simulink library "outp"  (R2021b)
(part 5 of 7)

  VBCM_CountAlarm_enum_Inproc : FVT_lib/outp/OverrideAndLimit  SystemSampleTime=-1  VariantActivationTime=update diagram  Latency=0  AutoFrameSizeCalculation=off
      link override Signal_Limit/_maxval: Value=KOUTP_CountAlarm_enum_maxval
      link override Signal_Limit/_minval: Value=KOUTP_CountAlarm_enum_minval
      link override Signal_Override/_ovrdflg: Value=KOUTP_CountAlarm_enum_ovrdflg
      link override Signal_Override/_ovrdval: Value=KOUTP_CountAlarm_enum_ovrdval
  VBCM_CrashDetd_flg_Inproc : FVT_lib/outp/OverrideAndLimit  SystemSampleTime=-1  VariantActivationTime=update diagram  Latency=0  AutoFrameSizeCalculation=off
      link override Signal_Limit/_maxval: Value=KOUTP_CrashDetd_flg_maxval
      link override Signal_Limit/_minval: Value=KOUTP_CrashDetd_flg_minval
      link override Signal_Override/_ovrdflg: Value=KOUTP_CrashDetd_flg_ovrdflg
      link override Signal_Override/_ovrdval: Value=KOUTP_CrashDetd_flg_ovrdval
  VBCM_DimSwSta_flg_Inproc : FVT_lib/outp/OverrideAndLimit  SystemSampleTime=-1  VariantActivationTime=update diagram  Latency=0  AutoFrameSizeCalculation=off
      link override Signal_Limit/_maxval: Value=KOUTP_DimSwSta_flg_maxval
      link override Signal_Limit/_minval: Value=KOUTP_DimSwSta_flg_minval
      link override Signal_Override/_ovrdflg: Value=KOUTP_DimSwSta_flg_ovrdflg
      link override Signal_Override/_ovrdval: Value=KOUTP_DimSwSta_flg_ovrdval
  VBCM_DimmerEN_flg_Inproc : FVT_lib/outp/OverrideAndLimit  SystemSampleTime=-1  VariantActivationTime=update diagram  Latency=0  AutoFrameSizeCalculation=off
      link override Signal_Limit/_maxval: Value=KOUTP_DimmerEN_flg_maxval
      link override Signal_Limit/_minval: Value=KOUTP_DimmerEN_flg_minval
      link override Signal_Override/_ovrdflg: Value=KOUTP_DimmerEN_flg_ovrdflg
      link override Signal_Override/_ovrdval: Value=KOUTP_DimmerEN_flg_ovrdval
  VBCM_Dimmer_pct_Inproc : FVT_lib/outp/OverrideAndLimit  SystemSampleTime=-1  VariantActivationTime=update diagram  Latency=0  AutoFrameSizeCalculation=off
      link override Signal_Limit/_maxval: Value=KOUTP_Dimmer_pct_maxval
      link override Signal_Limit/_minval: Value=KOUTP_Dimmer_pct_minval
      link override Signal_Override/_ovrdflg: Value=KOUTP_Dimmer_pct_ovrdflg
      link override Signal_Override/_ovrdval: Value=KOUTP_Dimmer_pct_ovrdval
  VBCM_DoorLockIND_flg_Inproc : FVT_lib/outp/OverrideAndLimit  SystemSampleTime=-1  VariantActivationTime=update diagram  Latency=0  AutoFrameSizeCalculation=off
      link override Signal_Limit/_maxval: Value=KOUTP_DoorLockIND_flg_maxval
      link override Signal_Limit/_minval: Value=KOUTP_DoorLockIND_flg_minval
      link override Signal_Override/_ovrdflg: Value=KOUTP_DoorLockIND_flg_ovrdflg
      link override Signal_Override/_ovrdval: Value=KOUTP_DoorLockIND_flg_ovrdval
  VBCM_DrDoorSW_flg_Inproc : FVT_lib/outp/OverrideAndLimit  SystemSampleTime=-1  VariantActivationTime=update diagram  Latency=0  AutoFrameSizeCalculation=off
      link override Signal_Limit/_maxval: Value=KOUTP_DrDoorSW_flg_maxval
      link override Signal_Limit/_minval: Value=KOUTP_DrDoorSW_flg_minval
      link override Signal_Override/_ovrdflg: Value=KOUTP_DrDoorSW_flg_ovrdflg
      link override Signal_Override/_ovrdval: Value=KOUTP_DrDoorSW_flg_ovrdval
  VBCM_FWasSwSta_enum_Inproc : FVT_lib/outp/OverrideAndLimit  SystemSampleTime=-1  VariantActivationTime=update diagram  Latency=0  AutoFrameSizeCalculation=off
      link override Signal_Limit/_maxval: Value=KOUTP_FWasSwSta_enum_maxval
      link override Signal_Limit/_minval: Value=KOUTP_FWasSwSta_enum_minval
      link override Signal_Override/_ovrdflg: Value=KOUTP_FWasSwSta_enum_ovrdflg
      link override Signal_Override/_ovrdval: Value=KOUTP_FWasSwSta_enum_ovrdval
  VBCM_FWipSwSta_enum_Inproc : FVT_lib/outp/OverrideAndLimit  SystemSampleTime=-1  VariantActivationTime=update diagram  Latency=0  AutoFrameSizeCalculation=off
      link override Signal_Limit/_maxval: Value=KOUTP_FWipSwSta_enum_maxval
      link override Signal_Limit/_minval: Value=KOUTP_FWipSwSta_enum_minval
      link override Signal_Override/_ovrdflg: Value=KOUTP_FWipSwSta_enum_ovrdflg
      link override Signal_Override/_ovrdval: Value=KOUTP_FWipSwSta_enum_ovrdval
  VBCM_FollowMe_flg_Inproc : FVT_lib/outp/OverrideAndLimit  SystemSampleTime=-1  VariantActivationTime=update diagram  Latency=0  AutoFrameSizeCalculation=off
      link override Signal_Limit/_maxval: Value=KOUTP_FollowMe_flg_maxval
      link override Signal_Limit/_minval: Value=KOUTP_FollowMe_flg_minval
      link override Signal_Override/_ovrdflg: Value=KOUTP_FollowMe_flg_ovrdflg
      link override Signal_Override/_ovrdval: Value=KOUTP_FollowMe_flg_ovrdval
  VBCM_FrChargingDoorCtrl_enum_Inproc : FVT_lib/outp/OverrideAndLimit  SystemSampleTime=-1  VariantActivationTime=update diagram  Latency=0  AutoFrameSizeCalculation=off
      link override Signal_Limit/_maxval: Value=KOUTP_FrChargingDoorCtrl_enum_maxval
      link override Signal_Limit/_minval: Value=KOUTP_FrChargingDoorCtrl_enum_minval
      link override Signal_Override/_ovrdflg: Value=KOUTP_FrChargingDoorCtrl_enum_ovrdflg
      link override Signal_Override/_ovrdval: Value=KOUTP_FrChargingDoorCtrl_enum_ovrdval
  VBCM_FrWiperH_flg_Inproc : FVT_lib/outp/OverrideAndLimit  SystemSampleTime=-1  VariantActivationTime=update diagram  Latency=0  AutoFrameSizeCalculation=off
      link override Signal_Limit/_maxval: Value=KOUTP_FrWiperH_flg_maxval
      link override Signal_Limit/_minval: Value=KOUTP_FrWiperH_flg_minval
      link override Signal_Override/_ovrdflg: Value=KOUTP_FrWiperH_flg_ovrdflg
      link override Signal_Override/_ovrdval: Value=KOUTP_FrWiperH_flg_ovrdval
  VBCM_FrWiperL_flg_Inproc : FVT_lib/outp/OverrideAndLimit  SystemSampleTime=-1  VariantActivationTime=update diagram  Latency=0  AutoFrameSizeCalculation=off
      link override Signal_Limit/_maxval: Value=KOUTP_FrWiperL_flg_maxval
      link override Signal_Limit/_minval: Value=KOUTP_FrWiperL_flg_minval
      link override Signal_Override/_ovrdflg: Value=KOUTP_FrWiperL_flg_ovrdflg
      link override Signal_Override/_ovrdval: Value=KOUTP_FrWiperL_flg_ovrdval
  VBCM_FuelDoorPos_flg_Inproc : FVT_lib/outp/OverrideAndLimit  SystemSampleTime=-1  VariantActivationTime=update diagram  Latency=0  AutoFrameSizeCalculation=off
      link override Signal_Limit/_maxval: Value=KOUTP_FuelDoorPos_flg_maxval
      link override Signal_Limit/_minval: Value=KOUTP_FuelDoorPos_flg_minval
      link override Signal_Override/_ovrdflg: Value=KOUTP_FuelDoorPos_flg_ovrdflg
      link override Signal_Override/_ovrdval: Value=KOUTP_FuelDoorPos_flg_ovrdval
  VBCM_HBeam_flg_Inproc : FVT_lib/outp/OverrideAndLimit  SystemSampleTime=-1  VariantActivationTime=update diagram  Latency=0  AutoFrameSizeCalculation=off
      link override Signal_Limit/_maxval: Value=KOUTP_HBeam_flg_maxval
      link override Signal_Limit/_minval: Value=KOUTP_HBeam_flg_minval
      link override Signal_Override/_ovrdflg: Value=KOUTP_HBeam_flg_ovrdflg
      link override Signal_Override/_ovrdval: Value=KOUTP_HBeam_flg_ovrdval
  VBCM_HazardIND_flg_Inproc : FVT_lib/outp/OverrideAndLimit  SystemSampleTime=-1  VariantActivationTime=update diagram  Latency=0  AutoFrameSizeCalculation=off
      link override Signal_Limit/_maxval: Value=KOUTP_HazardIND_flg_maxval
      link override Signal_Limit/_minval: Value=KOUTP_HazardIND_flg_minval
      link override Signal_Override/_ovrdflg: Value=KOUTP_HazardIND_flg_ovrdflg
      link override Signal_Override/_ovrdval: Value=KOUTP_HazardIND_flg_ovrdval
  VBCM_HazardSW_flg_Inproc : FVT_lib/outp/OverrideAndLimit  SystemSampleTime=-1  VariantActivationTime=update diagram  Latency=0  AutoFrameSizeCalculation=off
      link override Signal_Limit/_maxval: Value=KOUTP_HazardSW_flg_maxval
      link override Signal_Limit/_minval: Value=KOUTP_HazardSW_flg_minval
      link override Signal_Override/_ovrdflg: Value=KOUTP_HazardSW_flg_ovrdflg
      link override Signal_Override/_ovrdval: Value=KOUTP_HazardSW_flg_ovrdval
  VBCM_HoodSW_flg_Inproc : FVT_lib/outp/OverrideAndLimit  SystemSampleTime=-1  VariantActivationTime=update diagram  Latency=0  AutoFrameSizeCalculation=off
      link override Signal_Limit/_maxval: Value=KOUTP_HoodSW_flg_maxval
      link override Signal_Limit/_minval: Value=KOUTP_HoodSW_flg_minval
      link override Signal_Override/_ovrdflg: Value=KOUTP_HoodSW_flg_ovrdflg
      link override Signal_Override/_ovrdval: Value=KOUTP_HoodSW_flg_ovrdval
  VBCM_HornCtrl_flg_Inproc : FVT_lib/outp/OverrideAndLimit  SystemSampleTime=-1  VariantActivationTime=update diagram  Latency=0  AutoFrameSizeCalculation=off
      link override Signal_Limit/_maxval: Value=KOUTP_HornCtrl_flg_maxval
      link override Signal_Limit/_minval: Value=KOUTP_HornCtrl_flg_minval
      link override Signal_Override/_ovrdflg: Value=KOUTP_HornCtrl_flg_ovrdflg
      link override Signal_Override/_ovrdval: Value=KOUTP_HornCtrl_flg_ovrdval
  VBCM_IVIPTGUSStaSW_flg_Inproc : FVT_lib/outp/OverrideAndLimit  SystemSampleTime=-1  VariantActivationTime=update diagram  Latency=0  AutoFrameSizeCalculation=off
      link override Signal_Limit/_maxval: Value=KOUTP_IVIPTGUSStaSW_flg_maxval
      link override Signal_Limit/_minval: Value=KOUTP_IVIPTGUSStaSW_flg_minval
      link override Signal_Override/_ovrdflg: Value=KOUTP_IVIPTGUSStaSW_flg_ovrdflg
      link override Signal_Override/_ovrdval: Value=KOUTP_IVIPTGUSStaSW_flg_ovrdval
  VBCM_IVIRST_flg_Inproc : FVT_lib/outp/OverrideAndLimit  SystemSampleTime=-1  VariantActivationTime=update diagram  Latency=0  AutoFrameSizeCalculation=off
      link override Signal_Limit/_maxval: Value=KOUTP_IVIRST_flg_maxval
      link override Signal_Limit/_minval: Value=KOUTP_IVIRST_flg_minval
      link override Signal_Override/_ovrdflg: Value=KOUTP_IVIRST_flg_ovrdflg
      link override Signal_Override/_ovrdval: Value=KOUTP_IVIRST_flg_ovrdval
  VBCM_LBSD_flg_Inproc : FVT_lib/outp/OverrideAndLimit  SystemSampleTime=-1  VariantActivationTime=update diagram  Latency=0  AutoFrameSizeCalculation=off
      link override Signal_Limit/_maxval: Value=KOUTP_LBSD_flg_maxval
      link override Signal_Limit/_minval: Value=KOUTP_LBSD_flg_minval
      link override Signal_Override/_ovrdflg: Value=KOUTP_LBSD_flg_ovrdflg
      link override Signal_Override/_ovrdval: Value=KOUTP_LBSD_flg_ovrdval
  VBCM_LBeam_flg_Inproc : FVT_lib/outp/OverrideAndLimit  SystemSampleTime=-1  VariantActivationTime=update diagram  Latency=0  AutoFrameSizeCalculation=off
      link override Signal_Limit/_maxval: Value=KOUTP_LBeam_flg_maxval
      link override Signal_Limit/_minval: Value=KOUTP_LBeam_flg_minval
      link override Signal_Override/_ovrdflg: Value=KOUTP_LBeam_flg_ovrdflg
      link override Signal_Override/_ovrdval: Value=KOUTP_LBeam_flg_ovrdval
  VBCM_LDRL_flg_Inproc : FVT_lib/outp/OverrideAndLimit  SystemSampleTime=-1  VariantActivationTime=update diagram  Latency=0  AutoFrameSizeCalculation=off
      link override Signal_Limit/_maxval: Value=KOUTP_LDRL_flg_maxval
      link override Signal_Limit/_minval: Value=KOUTP_LDRL_flg_minval
      link override Signal_Override/_ovrdflg: Value=KOUTP_LDRL_flg_ovrdflg
      link override Signal_Override/_ovrdval: Value=KOUTP_LDRL_flg_ovrdval
  VBCM_LDrvCtrlCmd_pct_Inproc : FVT_lib/outp/OverrideAndLimit  SystemSampleTime=-1  VariantActivationTime=update diagram  Latency=0  AutoFrameSizeCalculation=off
      link override Signal_Limit/_maxval: Value=KOUTP_LDrvCtrlCmd_pct_maxval
      link override Signal_Limit/_minval: Value=KOUTP_LDrvCtrlCmd_pct_minval
      link override Signal_Override/_ovrdflg: Value=KOUTP_LDrvCtrlCmd_pct_ovrdflg
      link override Signal_Override/_ovrdval: Value=KOUTP_LDrvCtrlCmd_pct_ovrdval
  VBCM_LPasCtrlCmd_pct_Inproc : FVT_lib/outp/OverrideAndLimit  SystemSampleTime=-1  VariantActivationTime=update diagram  Latency=0  AutoFrameSizeCalculation=off
      link override Signal_Limit/_maxval: Value=KOUTP_LPasCtrlCmd_pct_maxval
      link override Signal_Limit/_minval: Value=KOUTP_LPasCtrlCmd_pct_minval
      link override Signal_Override/_ovrdflg: Value=KOUTP_LPasCtrlCmd_pct_ovrdflg
      link override Signal_Override/_ovrdval: Value=KOUTP_LPasCtrlCmd_pct_ovrdval
  VBCM_LRLDCtrlCmd_pct_Inproc : FVT_lib/outp/OverrideAndLimit  SystemSampleTime=-1  VariantActivationTime=update diagram  Latency=0  AutoFrameSizeCalculation=off
      link override Signal_Limit/_maxval: Value=KOUTP_LRLDCtrlCmd_pct_maxval
      link override Signal_Limit/_minval: Value=KOUTP_LRLDCtrlCmd_pct_minval
      link override Signal_Override/_ovrdflg: Value=KOUTP_LRLDCtrlCmd_pct_ovrdflg
      link override Signal_Override/_ovrdval: Value=KOUTP_LRLDCtrlCmd_pct_ovrdval
  VBCM_LRRDCtrlCmd_pct_Inproc : FVT_lib/outp/OverrideAndLimit  SystemSampleTime=-1  VariantActivationTime=update diagram  Latency=0  AutoFrameSizeCalculation=off
      link override Signal_Limit/_maxval: Value=KOUTP_LRRDCtrlCmd_pct_maxval
      link override Signal_Limit/_minval: Value=KOUTP_LRRDCtrlCmd_pct_minval
      link override Signal_Override/_ovrdflg: Value=KOUTP_LRRDCtrlCmd_pct_ovrdflg
      link override Signal_Override/_ovrdval: Value=KOUTP_LRRDCtrlCmd_pct_ovrdval
  VBCM_LTurnLP_flg_Inproc : FVT_lib/outp/OverrideAndLimit  SystemSampleTime=-1  VariantActivationTime=update diagram  Latency=0  AutoFrameSizeCalculation=off
      link override Signal_Limit/_maxval: Value=KOUTP_LTurnLP_flg_maxval
      link override Signal_Limit/_minval: Value=KOUTP_LTurnLP_flg_minval
      link override Signal_Override/_ovrdflg: Value=KOUTP_LTurnLP_flg_ovrdflg
      link override Signal_Override/_ovrdval: Value=KOUTP_LTurnLP_flg_ovrdval
  VBCM_LampPwr_flg_Inproc : FVT_lib/outp/OverrideAndLimit  SystemSampleTime=-1  VariantActivationTime=update diagram  Latency=0  AutoFrameSizeCalculation=off
      link override Signal_Limit/_maxval: Value=KOUTP_LampPwr_flg_maxval
      link override Signal_Limit/_minval: Value=KOUTP_LampPwr_flg_minval
      link override Signal_Override/_ovrdflg: Value=KOUTP_LampPwr_flg_ovrdflg
      link override Signal_Override/_ovrdval: Value=KOUTP_LampPwr_flg_ovrdval
  VBCM_LockAlarm_enum_Inproc : FVT_lib/outp/OverrideAndLimit  SystemSampleTime=-1  VariantActivationTime=update diagram  Latency=0  AutoFrameSizeCalculation=off
      link override Signal_Limit/_maxval: Value=KOUTP_LockAlarm_enum_maxval
      link override Signal_Limit/_minval: Value=KOUTP_LockAlarm_enum_minval
      link override Signal_Override/_ovrdflg: Value=KOUTP_LockAlarm_enum_ovrdflg
      link override Signal_Override/_ovrdval: Value=KOUTP_LockAlarm_enum_ovrdval
  VBCM_LockSetting_flg_Inproc : FVT_lib/outp/OverrideAndLimit  SystemSampleTime=-1  VariantActivationTime=update diagram  Latency=0  AutoFrameSizeCalculation=off
      link override Signal_Limit/_maxval: Value=KOUTP_LockSetting_flg_maxval
      link override Signal_Limit/_minval: Value=KOUTP_LockSetting_flg_minval
      link override Signal_Override/_ovrdflg: Value=KOUTP_LockSetting_flg_ovrdflg
      link override Signal_Override/_ovrdval: Value=KOUTP_LockSetting_flg_ovrdval
  VBCM_MFRDNBrightReq_pct_Inproc : FVT_lib/outp/OverrideAndLimit  SystemSampleTime=-1  VariantActivationTime=update diagram  Latency=0  AutoFrameSizeCalculation=off
      link override Signal_Limit/_maxval: Value=KOUTP_MFRDNBrightReq_pct_maxval
      link override Signal_Limit/_minval: Value=KOUTP_MFRDNBrightReq_pct_minval
      link override Signal_Override/_ovrdflg: Value=KOUTP_MFRDNBrightReq_pct_ovrdflg
      link override Signal_Override/_ovrdval: Value=KOUTP_MFRDNBrightReq_pct_ovrdval
  VBCM_MFSWTri_flg_Inproc : FVT_lib/outp/OverrideAndLimit  SystemSampleTime=-1  VariantActivationTime=update diagram  Latency=0  AutoFrameSizeCalculation=off
      link override Signal_Limit/_maxval: Value=KOUTP_MFSWTri_flg_maxval
      link override Signal_Limit/_minval: Value=KOUTP_MFSWTri_flg_minval
      link override Signal_Override/_ovrdflg: Value=KOUTP_MFSWTri_flg_ovrdflg
      link override Signal_Override/_ovrdval: Value=KOUTP_MFSWTri_flg_ovrdval
  VBCM_MirrorCtrl_enum_Inproc : FVT_lib/outp/OverrideAndLimit  SystemSampleTime=-1  VariantActivationTime=update diagram  Latency=0  AutoFrameSizeCalculation=off
      link override Signal_Limit/_maxval: Value=KOUTP_MirrorCtrl_enum_maxval
      link override Signal_Limit/_minval: Value=KOUTP_MirrorCtrl_enum_minval
      link override Signal_Override/_ovrdflg: Value=KOUTP_MirrorCtrl_enum_ovrdflg
      link override Signal_Override/_ovrdval: Value=KOUTP_MirrorCtrl_enum_ovrdval
  VBCM_MirrorDefog_flg_Inproc : FVT_lib/outp/OverrideAndLimit  SystemSampleTime=-1  VariantActivationTime=update diagram  Latency=0  AutoFrameSizeCalculation=off
      link override Signal_Limit/_maxval: Value=KOUTP_MirrorDefog_flg_maxval
      link override Signal_Limit/_minval: Value=KOUTP_MirrorDefog_flg_minval
      link override Signal_Override/_ovrdflg: Value=KOUTP_MirrorDefog_flg_ovrdflg
      link override Signal_Override/_ovrdval: Value=KOUTP_MirrorDefog_flg_ovrdval
  VBCM_MirrorFlodPos_flg_Inproc : FVT_lib/outp/OverrideAndLimit  SystemSampleTime=-1  VariantActivationTime=update diagram  Latency=0  AutoFrameSizeCalculation=off
      link override Signal_Limit/_maxval: Value=KOUTP_MirrorFlodPos_flg_maxval
      link override Signal_Limit/_minval: Value=KOUTP_MirrorFlodPos_flg_minval
      link override Signal_Override/_ovrdflg: Value=KOUTP_MirrorFlodPos_flg_ovrdflg
      link override Signal_Override/_ovrdval: Value=KOUTP_MirrorFlodPos_flg_ovrdval
  VBCM_PTGInnerSW2_enum_Inproc : FVT_lib/outp/OverrideAndLimit  SystemSampleTime=-1  VariantActivationTime=update diagram  Latency=0  AutoFrameSizeCalculation=off
      link override Signal_Limit/_maxval: Value=KOUTP_PTGInnerSW2_enum_maxval
      link override Signal_Limit/_minval: Value=KOUTP_PTGInnerSW2_enum_minval
      link override Signal_Override/_ovrdflg: Value=KOUTP_PTGInnerSW2_enum_ovrdflg
      link override Signal_Override/_ovrdval: Value=KOUTP_PTGInnerSW2_enum_ovrdval
  VBCM_PassSWSta_flg_Inproc : FVT_lib/outp/OverrideAndLimit  SystemSampleTime=-1  VariantActivationTime=update diagram  Latency=0  AutoFrameSizeCalculation=off
      link override Signal_Limit/_maxval: Value=KOUTP_PassSWSta_flg_maxval
      link override Signal_Limit/_minval: Value=KOUTP_PassSWSta_flg_minval
      link override Signal_Override/_ovrdflg: Value=KOUTP_PassSWSta_flg_ovrdflg
      link override Signal_Override/_ovrdval: Value=KOUTP_PassSWSta_flg_ovrdval
  VBCM_PosLamp_flg_Inproc : FVT_lib/outp/OverrideAndLimit  SystemSampleTime=-1  VariantActivationTime=update diagram  Latency=0  AutoFrameSizeCalculation=off
      link override Signal_Limit/_maxval: Value=KOUTP_PosLamp_flg_maxval
      link override Signal_Limit/_minval: Value=KOUTP_PosLamp_flg_minval
      link override Signal_Override/_ovrdflg: Value=KOUTP_PosLamp_flg_ovrdflg
      link override Signal_Override/_ovrdval: Value=KOUTP_PosLamp_flg_ovrdval
  VBCM_PsDoorSW_flg_Inproc : FVT_lib/outp/OverrideAndLimit  SystemSampleTime=-1  VariantActivationTime=update diagram  Latency=0  AutoFrameSizeCalculation=off
      link override Signal_Limit/_maxval: Value=KOUTP_PsDoorSW_flg_maxval
      link override Signal_Limit/_minval: Value=KOUTP_PsDoorSW_flg_minval
      link override Signal_Override/_ovrdflg: Value=KOUTP_PsDoorSW_flg_ovrdflg
      link override Signal_Override/_ovrdval: Value=KOUTP_PsDoorSW_flg_ovrdval
  VBCM_RBSD_flg_Inproc : FVT_lib/outp/OverrideAndLimit  SystemSampleTime=-1  VariantActivationTime=update diagram  Latency=0  AutoFrameSizeCalculation=off
      link override Signal_Limit/_maxval: Value=KOUTP_RBSD_flg_maxval
      link override Signal_Limit/_minval: Value=KOUTP_RBSD_flg_minval
      link override Signal_Override/_ovrdflg: Value=KOUTP_RBSD_flg_ovrdflg
      link override Signal_Override/_ovrdval: Value=KOUTP_RBSD_flg_ovrdval
  VBCM_RDRL_flg_Inproc : FVT_lib/outp/OverrideAndLimit  SystemSampleTime=-1  VariantActivationTime=update diagram  Latency=0  AutoFrameSizeCalculation=off
      link override Signal_Limit/_maxval: Value=KOUTP_RDRL_flg_maxval
      link override Signal_Limit/_minval: Value=KOUTP_RDRL_flg_minval
      link override Signal_Override/_ovrdflg: Value=KOUTP_RDRL_flg_ovrdflg
      link override Signal_Override/_ovrdval: Value=KOUTP_RDRL_flg_ovrdval
  VBCM_RLDoorSW_flg_Inproc : FVT_lib/outp/OverrideAndLimit  SystemSampleTime=-1  VariantActivationTime=update diagram  Latency=0  AutoFrameSizeCalculation=off
      link override Signal_Limit/_maxval: Value=KOUTP_RLDoorSW_flg_maxval
      link override Signal_Limit/_minval: Value=KOUTP_RLDoorSW_flg_minval
      link override Signal_Override/_ovrdflg: Value=KOUTP_RLDoorSW_flg_ovrdflg
      link override Signal_Override/_ovrdval: Value=KOUTP_RLDoorSW_flg_ovrdval
  VBCM_RRDoorSW_flg_Inproc : FVT_lib/outp/OverrideAndLimit  SystemSampleTime=-1  VariantActivationTime=update diagram  Latency=0  AutoFrameSizeCalculation=off
      link override Signal_Limit/_maxval: Value=KOUTP_RRDoorSW_flg_maxval
      link override Signal_Limit/_minval: Value=KOUTP_RRDoorSW_flg_minval
      link override Signal_Override/_ovrdflg: Value=KOUTP_RRDoorSW_flg_ovrdflg
      link override Signal_Override/_ovrdval: Value=KOUTP_RRDoorSW_flg_ovrdval
  VBCM_RTurnLP_flg_Inproc : FVT_lib/outp/OverrideAndLimit  SystemSampleTime=-1  VariantActivationTime=update diagram  Latency=0  AutoFrameSizeCalculation=off
      link override Signal_Limit/_maxval: Value=KOUTP_RTurnLP_flg_maxval
      link override Signal_Limit/_minval: Value=KOUTP_RTurnLP_flg_minval
      link override Signal_Override/_ovrdflg: Value=KOUTP_RTurnLP_flg_ovrdflg
      link override Signal_Override/_ovrdval: Value=KOUTP_RTurnLP_flg_ovrdval
  VBCM_ReverseLamp_flg_Inproc : FVT_lib/outp/OverrideAndLimit  SystemSampleTime=-1  VariantActivationTime=update diagram  Latency=0  AutoFrameSizeCalculation=off
      link override Signal_Limit/_maxval: Value=KOUTP_ReverseLamp_flg_maxval
      link override Signal_Limit/_minval: Value=KOUTP_ReverseLamp_flg_minval
      link override Signal_Override/_ovrdflg: Value=KOUTP_ReverseLamp_flg_ovrdflg
      link override Signal_Override/_ovrdval: Value=KOUTP_ReverseLamp_flg_ovrdval
  VBCM_RoomLampH_flg_Inproc : FVT_lib/outp/OverrideAndLimit  SystemSampleTime=-1  VariantActivationTime=update diagram  Latency=0  AutoFrameSizeCalculation=off
      link override Signal_Limit/_maxval: Value=KOUTP_RoomLampH_flg_maxval
      link override Signal_Limit/_minval: Value=KOUTP_RoomLampH_flg_minval
      link override Signal_Override/_ovrdflg: Value=KOUTP_RoomLampH_flg_ovrdflg
      link override Signal_Override/_ovrdval: Value=KOUTP_RoomLampH_flg_ovrdval
  VBCM_RoomLampL_flg_Inproc : FVT_lib/outp/OverrideAndLimit  SystemSampleTime=-1  VariantActivationTime=update diagram  Latency=0  AutoFrameSizeCalculation=off
      link override Signal_Limit/_maxval: Value=KOUTP_RoomLampL_flg_maxval
      link override Signal_Limit/_minval: Value=KOUTP_RoomLampL_flg_minval
      link override Signal_Override/_ovrdflg: Value=KOUTP_RoomLampL_flg_ovrdflg
      link override Signal_Override/_ovrdval: Value=KOUTP_RoomLampL_flg_ovrdval
  VBCM_RoomLampMode_flg_Inproc : FVT_lib/outp/OverrideAndLimit  SystemSampleTime=-1  VariantActivationTime=update diagram  Latency=0  AutoFrameSizeCalculation=off
      link override Signal_Limit/_maxval: Value=KOUTP_RoomLampMode_flg_maxval
      link override Signal_Limit/_minval: Value=KOUTP_RoomLampMode_flg_minval
      link override Signal_Override/_ovrdflg: Value=KOUTP_RoomLampMode_flg_ovrdflg
      link override Signal_Override/_ovrdval: Value=KOUTP_RoomLampMode_flg_ovrdval
  VBCM_RrChargingDoorCtrl_enum_Inproc : FVT_lib/outp/OverrideAndLimit  SystemSampleTime=-1  VariantActivationTime=update diagram  Latency=0  AutoFrameSizeCalculation=off
      link override Signal_Limit/_maxval: Value=KOUTP_RrChargingDoorCtrl_enum_maxval
      link override Signal_Limit/_minval: Value=KOUTP_RrChargingDoorCtrl_enum_minval
      link override Signal_Override/_ovrdflg: Value=KOUTP_RrChargingDoorCtrl_enum_ovrdflg
      link override Signal_Override/_ovrdval: Value=KOUTP_RrChargingDoorCtrl_enum_ovrdval
  VBCM_RrDefog_flg_Inproc : FVT_lib/outp/OverrideAndLimit  SystemSampleTime=-1  VariantActivationTime=update diagram  Latency=0  AutoFrameSizeCalculation=off
      link override Signal_Limit/_maxval: Value=KOUTP_RrDefog_flg_maxval
      link override Signal_Limit/_minval: Value=KOUTP_RrDefog_flg_minval
      link override Signal_Override/_ovrdflg: Value=KOUTP_RrDefog_flg_ovrdflg
      link override Signal_Override/_ovrdval: Value=KOUTP_RrDefog_flg_ovrdval
  VBCM_RrFogLamp_flg_Inproc : FVT_lib/outp/OverrideAndLimit  SystemSampleTime=-1  VariantActivationTime=update diagram  Latency=0  AutoFrameSizeCalculation=off
      link override Signal_Limit/_maxval: Value=KOUTP_RrFogLamp_flg_maxval
      link override Signal_Limit/_minval: Value=KOUTP_RrFogLamp_flg_minval
      link override Signal_Override/_ovrdflg: Value=KOUTP_RrFogLamp_flg_ovrdflg
      link override Signal_Override/_ovrdval: Value=KOUTP_RrFogLamp_flg_ovrdval
  VBCM_RrWiper_flg_Inproc : FVT_lib/outp/OverrideAndLimit  SystemSampleTime=-1  VariantActivationTime=update diagram  Latency=0  AutoFrameSizeCalculation=off
      link override Signal_Limit/_maxval: Value=KOUTP_RrWiper_flg_maxval
      link override Signal_Limit/_minval: Value=KOUTP_RrWiper_flg_minval
      link override Signal_Override/_ovrdflg: Value=KOUTP_RrWiper_flg_ovrdflg
      link override Signal_Override/_ovrdval: Value=KOUTP_RrWiper_flg_ovrdval
  VBCM_SPTGDet_flg_Inproc : FVT_lib/outp/OverrideAndLimit  SystemSampleTime=-1  VariantActivationTime=update diagram  Latency=0  AutoFrameSizeCalculation=off
      link override Signal_Limit/_maxval: Value=KOUTP_SPTGDet_flg_maxval
      link override Signal_Limit/_minval: Value=KOUTP_SPTGDet_flg_minval
      link override Signal_Override/_ovrdflg: Value=KOUTP_SPTGDet_flg_ovrdflg
      link override Signal_Override/_ovrdval: Value=KOUTP_SPTGDet_flg_ovrdval
  VBCM_TailgateHDSW_flg_Inproc : FVT_lib/outp/OverrideAndLimit  SystemSampleTime=-1  VariantActivationTime=update diagram  Latency=0  AutoFrameSizeCalculation=off
      link override Signal_Limit/_maxval: Value=KOUTP_TailgateHDSW_flg_maxval
      link override Signal_Limit/_minval: Value=KOUTP_TailgateHDSW_flg_minval
      link override Signal_Override/_ovrdflg: Value=KOUTP_TailgateHDSW_flg_ovrdflg
      link override Signal_Override/_ovrdval: Value=KOUTP_TailgateHDSW_flg_ovrdval
  VBCM_TailgateRemote_enum_Inproc : FVT_lib/outp/OverrideAndLimit  SystemSampleTime=-1  VariantActivationTime=update diagram  Latency=0  AutoFrameSizeCalculation=off
      link override Signal_Limit/_maxval: Value=KOUTP_TailgateRemote_enum_maxval
      link override Signal_Limit/_minval: Value=KOUTP_TailgateRemote_enum_minval
      link override Signal_Override/_ovrdflg: Value=KOUTP_TailgateRemote_enum_ovrdflg
      link override Signal_Override/_ovrdval: Value=KOUTP_TailgateRemote_enum_ovrdval
  VBCM_TailgateSW_flg_Inproc : FVT_lib/outp/OverrideAndLimit  SystemSampleTime=-1  VariantActivationTime=update diagram  Latency=0  AutoFrameSizeCalculation=off
      link override Signal_Limit/_maxval: Value=KOUTP_TailgateSW_flg_maxval
      link override Signal_Limit/_minval: Value=KOUTP_TailgateSW_flg_minval
      link override Signal_Override/_ovrdflg: Value=KOUTP_TailgateSW_flg_ovrdflg
      link override Signal_Override/_ovrdval: Value=KOUTP_TailgateSW_flg_ovrdval
  VBCM_TrunkRel_flg_Inproc : FVT_lib/outp/OverrideAndLimit  SystemSampleTime=-1  VariantActivationTime=update diagram  Latency=0  AutoFrameSizeCalculation=off
      link override Signal_Limit/_maxval: Value=KOUTP_TrunkRel_flg_maxval
      link override Signal_Limit/_minval: Value=KOUTP_TrunkRel_flg_minval
      link override Signal_Override/_ovrdflg: Value=KOUTP_TrunkRel_flg_ovrdflg
      link override Signal_Override/_ovrdval: Value=KOUTP_TrunkRel_flg_ovrdval
  VBCM_TurnSwSta_enum_Inproc : FVT_lib/outp/OverrideAndLimit  SystemSampleTime=-1  VariantActivationTime=update diagram  Latency=0  AutoFrameSizeCalculation=off
      link override Signal_Limit/_maxval: Value=KOUTP_TurnSwSta_enum_maxval
      link override Signal_Limit/_minval: Value=KOUTP_TurnSwSta_enum_minval
      link override Signal_Override/_ovrdflg: Value=KOUTP_TurnSwSta_enum_ovrdflg
      link override Signal_Override/_ovrdval: Value=KOUTP_TurnSwSta_enum_ovrdval
  VBCM_UserNow_enum_Inproc : FVT_lib/outp/OverrideAndLimit  SystemSampleTime=-1  VariantActivationTime=update diagram  Latency=0  AutoFrameSizeCalculation=off
      link override Signal_Limit/_maxval: Value=KOUTP_UserNow_enum_maxval
      link override Signal_Limit/_minval: Value=KOUTP_UserNow_enum_minval
      link override Signal_Override/_ovrdflg: Value=KOUTP_UserNow_enum_ovrdflg
      link override Signal_Override/_ovrdval: Value=KOUTP_UserNow_enum_ovrdval
  VBCM_WasherCtrl_enum_Inproc : FVT_lib/outp/OverrideAndLimit  SystemSampleTime=-1  VariantActivationTime=update diagram  Latency=0  AutoFrameSizeCalculation=off
      link override Signal_Limit/_maxval: Value=KOUTP_WasherCtrl_enum_maxval
      link override Signal_Limit/_minval: Value=KOUTP_WasherCtrl_enum_minval
      link override Signal_Override/_ovrdflg: Value=KOUTP_WasherCtrl_enum_ovrdflg
      link override Signal_Override/_ovrdval: Value=KOUTP_WasherCtrl_enum_ovrdval
  VBCM_WiperFixMode_flg_Inproc : FVT_lib/outp/OverrideAndLimit  SystemSampleTime=-1  VariantActivationTime=update diagram  Latency=0  AutoFrameSizeCalculation=off
      link override Signal_Limit/_maxval: Value=KOUTP_WiperFixMode_flg_maxval
      link override Signal_Limit/_minval: Value=KOUTP_WiperFixMode_flg_minval
      link override Signal_Override/_ovrdflg: Value=KOUTP_WiperFixMode_flg_ovrdflg
      link override Signal_Override/_ovrdval: Value=KOUTP_WiperFixMode_flg_ovrdval
  VBCM_fUnlockSingle_flg_Inproc : FVT_lib/outp/OverrideAndLimit  SystemSampleTime=-1  VariantActivationTime=update diagram  Latency=0  AutoFrameSizeCalculation=off
      link override Signal_Limit/_maxval: Value=KOUTP_fUnlockSingle_flg_maxval
      link override Signal_Limit/_minval: Value=KOUTP_fUnlockSingle_flg_minval
      link override Signal_Override/_ovrdflg: Value=KOUTP_fUnlockSingle_flg_ovrdflg
      link override Signal_Override/_ovrdval: Value=KOUTP_fUnlockSingle_flg_ovrdval
  VDHP_ActAPSPosn_pct_Inproc : FVT_lib/outp/OverrideAndLimit  SystemSampleTime=-1  VariantActivationTime=update diagram  Latency=0  AutoFrameSizeCalculation=off
      link override Signal_Limit/_maxval: Value=KOUTP_ActAPSPosn_pct_maxval
      link override Signal_Limit/_minval: Value=KOUTP_ActAPSPosn_pct_minval
      link override Signal_Override/_ovrdflg: Value=KOUTP_ActAPSPosn_pct_ovrdflg
      link override Signal_Override/_ovrdval: Value=KOUTP_ActAPSPosn_pct_ovrdval
  VDHP_EAPS1MIN_pct_Inproc : FVT_lib/outp/OverrideAndLimit  SystemSampleTime=-1  VariantActivationTime=update diagram  Latency=0  AutoFrameSizeCalculation=off
      link override Signal_Limit/_maxval: Value=KOUTP_EAPS1MIN_pct_maxval
      link override Signal_Limit/_minval: Value=KOUTP_EAPS1MIN_pct_minval
      link override Signal_Override/_ovrdflg: Value=KOUTP_EAPS1MIN_pct_ovrdflg
      link override Signal_Override/_ovrdval: Value=KOUTP_EAPS1MIN_pct_ovrdval
  VDHP_EAPS2MIN_pct_Inproc : FVT_lib/outp/OverrideAndLimit  SystemSampleTime=-1  VariantActivationTime=update diagram  Latency=0  AutoFrameSizeCalculation=off
      link override Signal_Limit/_maxval: Value=KOUTP_EAPS2MIN_pct_maxval
      link override Signal_Limit/_minval: Value=KOUTP_EAPS2MIN_pct_minval
      link override Signal_Override/_ovrdflg: Value=KOUTP_EAPS2MIN_pct_ovrdflg
      link override Signal_Override/_ovrdval: Value=KOUTP_EAPS2MIN_pct_ovrdval
  VDKC_DKCAuthSta_enum_Inproc : FVT_lib/outp/OverrideAndLimit  SystemSampleTime=-1  VariantActivationTime=update diagram  Latency=0  AutoFrameSizeCalculation=off
      link override Signal_Limit/_maxval: Value=KOUTP_DKCAuthSta_enum_maxval
      link override Signal_Limit/_minval: Value=KOUTP_DKCAuthSta_enum_minval
      link override Signal_Override/_ovrdflg: Value=KOUTP_DKCAuthSta_enum_ovrdflg
      link override Signal_Override/_ovrdval: Value=KOUTP_DKCAuthSta_enum_ovrdval
  VDKC_DKCTimeSN_cnt_Inproc : FVT_lib/outp/OverrideAndLimit  SystemSampleTime=-1  VariantActivationTime=update diagram  Latency=0  AutoFrameSizeCalculation=off
      link override Signal_Limit/_maxval: Value=KOUTP_DKCTimeSN_cnt_maxval
      link override Signal_Limit/_minval: Value=KOUTP_DKCTimeSN_cnt_minval
      link override Signal_Override/_ovrdflg: Value=KOUTP_DKCTimeSN_cnt_ovrdflg
      link override Signal_Override/_ovrdval: Value=KOUTP_DKCTimeSN_cnt_ovrdval
  VDSC_DISCButtSta_flg_Inproc : FVT_lib/outp/OverrideAndLimit  SystemSampleTime=-1  VariantActivationTime=update diagram  Latency=0  AutoFrameSizeCalculation=off
      link override Signal_Limit/_maxval: Value=KOUTP_DISCButtSta_flg_maxval
      link override Signal_Limit/_minval: Value=KOUTP_DISCButtSta_flg_minval
      link override Signal_Override/_ovrdflg: Value=KOUTP_DISCButtSta_flg_ovrdflg
      link override Signal_Override/_ovrdval: Value=KOUTP_DISCButtSta_flg_ovrdval
  VDSC_DISCSta_enum_Inproc : FVT_lib/outp/OverrideAndLimit  SystemSampleTime=-1  VariantActivationTime=update diagram  Latency=0  AutoFrameSizeCalculation=off
      link override Signal_Limit/_maxval: Value=KOUTP_DISCSta_enum_maxval
      link override Signal_Limit/_minval: Value=KOUTP_DISCSta_enum_minval
      link override Signal_Override/_ovrdflg: Value=KOUTP_DISCSta_enum_ovrdflg
      link override Signal_Override/_ovrdval: Value=KOUTP_DISCSta_enum_ovrdval
  VDSC_DISCTargetSpd_kph_Inproc : FVT_lib/outp/OverrideAndLimit  SystemSampleTime=-1  VariantActivationTime=update diagram  Latency=0  AutoFrameSizeCalculation=off
      link override Signal_Limit/_maxval: Value=KOUTP_DISCTargetSpd_kph_maxval
      link override Signal_Limit/_minval: Value=KOUTP_DISCTargetSpd_kph_minval
      link override Signal_Override/_ovrdflg: Value=KOUTP_DISCTargetSpd_kph_ovrdflg
      link override Signal_Override/_ovrdval: Value=KOUTP_DISCTargetSpd_kph_ovrdval
  VDSC_DISCTurn_flg_Inproc : FVT_lib/outp/OverrideAndLimit  SystemSampleTime=-1  VariantActivationTime=update diagram  Latency=0  AutoFrameSizeCalculation=off
      link override Signal_Limit/_maxval: Value=KOUTP_DISCTurn_flg_maxval
      link override Signal_Limit/_minval: Value=KOUTP_DISCTurn_flg_minval
      link override Signal_Override/_ovrdflg: Value=KOUTP_DISCTurn_flg_ovrdflg
      link override Signal_Override/_ovrdval: Value=KOUTP_DISCTurn_flg_ovrdval
  VNMM_ActiveWU_flg_Inproc : FVT_lib/outp/OverrideAndLimit  SystemSampleTime=-1  VariantActivationTime=update diagram  Latency=0  AutoFrameSizeCalculation=off
      link override Signal_Limit/_maxval: Value=KOUTP_ActiveWU_flg_maxval
      link override Signal_Limit/_minval: Value=KOUTP_ActiveWU_flg_minval
      link override Signal_Override/_ovrdflg: Value=KOUTP_ActiveWU_flg_ovrdflg
      link override Signal_Override/_ovrdval: Value=KOUTP_ActiveWU_flg_ovrdval
  VNMM_AllCANTxReq_flg_Inproc : FVT_lib/outp/OverrideAndLimit  SystemSampleTime=-1  VariantActivationTime=update diagram  Latency=0  AutoFrameSizeCalculation=off
      link override Signal_Limit/_maxval: Value=KOUTP_AllCANTxReq_flg_maxval
      link override Signal_Limit/_minval: Value=KOUTP_AllCANTxReq_flg_minval
      link override Signal_Override/_ovrdflg: Value=KOUTP_AllCANTxReq_flg_ovrdflg
      link override Signal_Override/_ovrdval: Value=KOUTP_AllCANTxReq_flg_ovrdval
  VNMM_Awake_enum_Inproc : FVT_lib/outp/OverrideAndLimit  SystemSampleTime=-1  VariantActivationTime=update diagram  Latency=0  AutoFrameSizeCalculation=off
      link override Signal_Limit/_maxval: Value=KOUTP_Awake_enum_maxval
      link override Signal_Limit/_minval: Value=KOUTP_Awake_enum_minval
      link override Signal_Override/_ovrdflg: Value=KOUTP_Awake_enum_ovrdflg
      link override Signal_Override/_ovrdval: Value=KOUTP_Awake_enum_ovrdval
  VNMM_CSB_flg_Inproc : FVT_lib/outp/OverrideAndLimit  SystemSampleTime=-1  VariantActivationTime=update diagram  Latency=0  AutoFrameSizeCalculation=off
      link override Signal_Limit/_maxval: Value=KOUTP_CSB_flg_maxval
      link override Signal_Limit/_minval: Value=KOUTP_CSB_flg_minval
      link override Signal_Override/_ovrdflg: Value=KOUTP_CSB_flg_ovrdflg
      link override Signal_Override/_ovrdval: Value=KOUTP_CSB_flg_ovrdval
  VNMM_ErrorState_enum_Inproc : FVT_lib/outp/OverrideAndLimit  SystemSampleTime=-1  VariantActivationTime=update diagram  Latency=0  AutoFrameSizeCalculation=off
      link override Signal_Limit/_maxval: Value=KOUTP_ErrorState_enum_maxval
      link override Signal_Limit/_minval: Value=KOUTP_ErrorState_enum_minval
      link override Signal_Override/_ovrdflg: Value=KOUTP_ErrorState_enum_ovrdflg
      link override Signal_Override/_ovrdval: Value=KOUTP_ErrorState_enum_ovrdval
  VNMM_NMmTxReq_flg_Inproc : FVT_lib/outp/OverrideAndLimit  SystemSampleTime=-1  VariantActivationTime=update diagram  Latency=0  AutoFrameSizeCalculation=off
      link override Signal_Limit/_maxval: Value=KOUTP_NMmTxReq_flg_maxval
      link override Signal_Limit/_minval: Value=KOUTP_NMmTxReq_flg_minval
      link override Signal_Override/_ovrdflg: Value=KOUTP_NMmTxReq_flg_ovrdflg
      link override Signal_Override/_ovrdval: Value=KOUTP_NMmTxReq_flg_ovrdval
  VNMM_NetworkReq_flg_Inproc : FVT_lib/outp/OverrideAndLimit  SystemSampleTime=-1  VariantActivationTime=update diagram  Latency=0  AutoFrameSizeCalculation=off
      link override Signal_Limit/_maxval: Value=KOUTP_NetworkReq_flg_maxval
      link override Signal_Limit/_minval: Value=KOUTP_NetworkReq_flg_minval
      link override Signal_Override/_ovrdflg: Value=KOUTP_NetworkReq_flg_ovrdflg
      link override Signal_Override/_ovrdval: Value=KOUTP_NetworkReq_flg_ovrdval
  VNMM_NodeID_enum_Inproc : FVT_lib/outp/OverrideAndLimit  SystemSampleTime=-1  VariantActivationTime=update diagram  Latency=0  AutoFrameSizeCalculation=off
      link override Signal_Limit/_maxval: Value=KOUTP_NodeID_enum_maxval
      link override Signal_Limit/_minval: Value=KOUTP_NodeID_enum_minval
      link override Signal_Override/_ovrdflg: Value=KOUTP_NodeID_enum_ovrdflg
      link override Signal_Override/_ovrdval: Value=KOUTP_NodeID_enum_ovrdval
  VNMM_PNI_flg_Inproc : FVT_lib/outp/OverrideAndLimit  SystemSampleTime=-1  VariantActivationTime=update diagram  Latency=0  AutoFrameSizeCalculation=off
      link override Signal_Limit/_maxval: Value=KOUTP_PNI_flg_maxval
      link override Signal_Limit/_minval: Value=KOUTP_PNI_flg_minval
      link override Signal_Override/_ovrdflg: Value=KOUTP_PNI_flg_ovrdflg
      link override Signal_Override/_ovrdval: Value=KOUTP_PNI_flg_ovrdval
  VNMM_RptMsgReq_flg_Inproc : FVT_lib/outp/OverrideAndLimit  SystemSampleTime=-1  VariantActivationTime=update diagram  Latency=0  AutoFrameSizeCalculation=off
      link override Signal_Limit/_maxval: Value=KOUTP_RptMsgReq_flg_maxval
      link override Signal_Limit/_minval: Value=KOUTP_RptMsgReq_flg_minval
      link override Signal_Override/_ovrdflg: Value=KOUTP_RptMsgReq_flg_ovrdflg
      link override Signal_Override/_ovrdval: Value=KOUTP_RptMsgReq_flg_ovrdval
  VNMM_SysNMmSta_enum_Inproc : FVT_lib/outp/OverrideAndLimit  SystemSampleTime=-1  VariantActivationTime=update diagram  Latency=0  AutoFrameSizeCalculation=off
      link override Signal_Limit/_maxval: Value=KOUTP_SysNMmSta_enum_maxval
      link override Signal_Limit/_minval: Value=KOUTP_SysNMmSta_enum_minval
      link override Signal_Override/_ovrdflg: Value=KOUTP_SysNMmSta_enum_ovrdflg
      link override Signal_Override/_ovrdval: Value=KOUTP_SysNMmSta_enum_ovrdval
  VNMM_WakeUp_enum_Inproc : FVT_lib/outp/OverrideAndLimit  SystemSampleTime=-1  VariantActivationTime=update diagram  Latency=0  AutoFrameSizeCalculation=off
      link override Signal_Limit/_maxval: Value=KOUTP_WakeUp_enum_maxval
      link override Signal_Limit/_minval: Value=KOUTP_WakeUp_enum_minval
      link override Signal_Override/_ovrdflg: Value=KOUTP_WakeUp_enum_ovrdflg
      link override Signal_Override/_ovrdval: Value=KOUTP_WakeUp_enum_ovrdval
  VPMM_ActiveDischargeReq_flg_Inproc : FVT_lib/outp/OverrideAndLimit  SystemSampleTime=-1  VariantActivationTime=update diagram  Latency=0  AutoFrameSizeCalculation=off
      link override Signal_Limit/_maxval: Value=KOUTP_ActiveDischargeReq_flg_maxval
      link override Signal_Limit/_minval: Value=KOUTP_ActiveDischargeReq_flg_minval
      link override Signal_Override/_ovrdflg: Value=KOUTP_ActiveDischargeReq_flg_ovrdflg
      link override Signal_Override/_ovrdval: Value=KOUTP_ActiveDischargeReq_flg_ovrdval
  VPMM_CtrlDrPwrStbA2_flg_Inproc : FVT_lib/outp/OverrideAndLimit  SystemSampleTime=-1  VariantActivationTime=update diagram  Latency=0  AutoFrameSizeCalculation=off
      link override Signal_Limit/_maxval: Value=KOUTP_CtrlDrPwrStbA2_flg_maxval
      link override Signal_Limit/_minval: Value=KOUTP_CtrlDrPwrStbA2_flg_minval
      link override Signal_Override/_ovrdflg: Value=KOUTP_CtrlDrPwrStbA2_flg_ovrdflg
      link override Signal_Override/_ovrdval: Value=KOUTP_CtrlDrPwrStbA2_flg_ovrdval
  VPMM_CtrlFrBMSCCUCIR_flg_Inproc : FVT_lib/outp/OverrideAndLimit  SystemSampleTime=-1  VariantActivationTime=update diagram  Latency=0  AutoFrameSizeCalculation=off
      link override Signal_Limit/_maxval: Value=KOUTP_CtrlFrBMSCCUCIR_flg_maxval
      link override Signal_Limit/_minval: Value=KOUTP_CtrlFrBMSCCUCIR_flg_minval
      link override Signal_Override/_ovrdflg: Value=KOUTP_CtrlFrBMSCCUCIR_flg_ovrdflg
      link override Signal_Override/_ovrdval: Value=KOUTP_CtrlFrBMSCCUCIR_flg_ovrdval
  VPMM_CtrlFrEDUINVERTER_flg_Inproc : FVT_lib/outp/OverrideAndLimit  SystemSampleTime=-1  VariantActivationTime=update diagram  Latency=0  AutoFrameSizeCalculation=off
      link override Signal_Limit/_maxval: Value=KOUTP_CtrlFrEDUINVERTER_flg_maxval
      link override Signal_Limit/_minval: Value=KOUTP_CtrlFrEDUINVERTER_flg_minval
      link override Signal_Override/_ovrdflg: Value=KOUTP_CtrlFrEDUINVERTER_flg_ovrdflg
      link override Signal_Override/_ovrdval: Value=KOUTP_CtrlFrEDUINVERTER_flg_ovrdval
  VPMM_CtrlFrPwrStbA1P_flg_Inproc : FVT_lib/outp/OverrideAndLimit  SystemSampleTime=-1  VariantActivationTime=update diagram  Latency=0  AutoFrameSizeCalculation=off
      link override Signal_Limit/_maxval: Value=KOUTP_CtrlFrPwrStbA1P_flg_maxval
      link override Signal_Limit/_minval: Value=KOUTP_CtrlFrPwrStbA1P_flg_minval
      link override Signal_Override/_ovrdflg: Value=KOUTP_CtrlFrPwrStbA1P_flg_ovrdflg
      link override Signal_Override/_ovrdval: Value=KOUTP_CtrlFrPwrStbA1P_flg_ovrdval
  VPMM_CtrlFrRC1_flg_Inproc : FVT_lib/outp/OverrideAndLimit  SystemSampleTime=-1  VariantActivationTime=update diagram  Latency=0  AutoFrameSizeCalculation=off
      link override Signal_Limit/_maxval: Value=KOUTP_CtrlFrRC1_flg_maxval
      link override Signal_Limit/_minval: Value=KOUTP_CtrlFrRC1_flg_minval
      link override Signal_Override/_ovrdflg: Value=KOUTP_CtrlFrRC1_flg_ovrdflg
      link override Signal_Override/_ovrdval: Value=KOUTP_CtrlFrRC1_flg_ovrdval
  VPMM_DCDCEnaReq_flg_Inproc : FVT_lib/outp/OverrideAndLimit  SystemSampleTime=-1  VariantActivationTime=update diagram  Latency=0  AutoFrameSizeCalculation=off
      link override Signal_Limit/_maxval: Value=KOUTP_DCDCEnaReq_flg_maxval
      link override Signal_Limit/_minval: Value=KOUTP_DCDCEnaReq_flg_minval
      link override Signal_Override/_ovrdflg: Value=KOUTP_DCDCEnaReq_flg_ovrdflg
      link override Signal_Override/_ovrdval: Value=KOUTP_DCDCEnaReq_flg_ovrdval
  VPMM_DCDCVoltSetpoint_V_Inproc : FVT_lib/outp/OverrideAndLimit  SystemSampleTime=-1  VariantActivationTime=update diagram  Latency=0  AutoFrameSizeCalculation=off
      link override Signal_Limit/_maxval: Value=KOUTP_DCDCVoltSetpoint_V_maxval
      link override Signal_Limit/_minval: Value=KOUTP_DCDCVoltSetpoint_V_minval
      link override Signal_Override/_ovrdflg: Value=KOUTP_DCDCVoltSetpoint_V_ovrdflg
      link override Signal_Override/_ovrdval: Value=KOUTP_DCDCVoltSetpoint_V_ovrdval
  VPMM_DrSeatSta_enum_Inproc : FVT_lib/outp/OverrideAndLimit  SystemSampleTime=-1  VariantActivationTime=update diagram  Latency=0  AutoFrameSizeCalculation=off
      link override Signal_Limit/_maxval: Value=KOUTP_DrSeatSta_enum_maxval
      link override Signal_Limit/_minval: Value=KOUTP_DrSeatSta_enum_minval
      link override Signal_Override/_ovrdflg: Value=KOUTP_DrSeatSta_enum_ovrdflg
      link override Signal_Override/_ovrdval: Value=KOUTP_DrSeatSta_enum_ovrdval
  VPMM_DrivetrainSelect_enum_Inproc : FVT_lib/outp/OverrideAndLimit  SystemSampleTime=-1  VariantActivationTime=update diagram  Latency=0  AutoFrameSizeCalculation=off
      link override Signal_Limit/_maxval: Value=KOUTP_DrivetrainSelect_enum_maxval
      link override Signal_Limit/_minval: Value=KOUTP_DrivetrainSelect_enum_minval
      link override Signal_Override/_ovrdflg: Value=KOUTP_DrivetrainSelect_enum_ovrdflg
      link override Signal_Override/_ovrdval: Value=KOUTP_DrivetrainSelect_enum_ovrdval
  VPMM_EvccAplusPwrUpReq_flg_Inproc : FVT_lib/outp/OverrideAndLimit  SystemSampleTime=-1  VariantActivationTime=update diagram  Latency=0  AutoFrameSizeCalculation=off
      link override Signal_Limit/_maxval: Value=KOUTP_EvccAplusPwrUpReq_flg_maxval
      link override Signal_Limit/_minval: Value=KOUTP_EvccAplusPwrUpReq_flg_minval
      link override Signal_Override/_ovrdflg: Value=KOUTP_EvccAplusPwrUpReq_flg_ovrdflg
      link override Signal_Override/_ovrdval: Value=KOUTP_EvccAplusPwrUpReq_flg_ovrdval
  VPMM_FDADC12VDetAvg_mV_Inproc : FVT_lib/outp/OverrideAndLimit  SystemSampleTime=-1  VariantActivationTime=update diagram  Latency=0  AutoFrameSizeCalculation=off
      link override Signal_Limit/_maxval: Value=KOUTP_FDADC12VDetAvg_mV_maxval
      link override Signal_Limit/_minval: Value=KOUTP_FDADC12VDetAvg_mV_minval
      link override Signal_Override/_ovrdflg: Value=KOUTP_FDADC12VDetAvg_mV_ovrdflg
      link override Signal_Override/_ovrdval: Value=KOUTP_FDADC12VDetAvg_mV_ovrdval
  VPMM_FrMCUEnaReq_flg_Inproc : FVT_lib/outp/OverrideAndLimit  SystemSampleTime=-1  VariantActivationTime=update diagram  Latency=0  AutoFrameSizeCalculation=off
      link override Signal_Limit/_maxval: Value=KOUTP_FrMCUEnaReq_flg_maxval
      link override Signal_Limit/_minval: Value=KOUTP_FrMCUEnaReq_flg_minval
      link override Signal_Override/_ovrdflg: Value=KOUTP_FrMCUEnaReq_flg_ovrdflg
      link override Signal_Override/_ovrdval: Value=KOUTP_FrMCUEnaReq_flg_ovrdval
  VPMM_HVBatCnctReq_flg_Inproc : FVT_lib/outp/OverrideAndLimit  SystemSampleTime=-1  VariantActivationTime=update diagram  Latency=0  AutoFrameSizeCalculation=off
      link override Signal_Limit/_maxval: Value=KOUTP_HVBatCnctReq_flg_maxval
      link override Signal_Limit/_minval: Value=KOUTP_HVBatCnctReq_flg_minval
      link override Signal_Override/_ovrdflg: Value=KOUTP_HVBatCnctReq_flg_ovrdflg
      link override Signal_Override/_ovrdval: Value=KOUTP_HVBatCnctReq_flg_ovrdval
  VPMM_HVPwrSta_flg_Inproc : FVT_lib/outp/OverrideAndLimit  SystemSampleTime=-1  VariantActivationTime=update diagram  Latency=0  AutoFrameSizeCalculation=off
      link override Signal_Limit/_maxval: Value=KOUTP_HVPwrSta_flg_maxval
      link override Signal_Limit/_minval: Value=KOUTP_HVPwrSta_flg_minval
      link override Signal_Override/_ovrdflg: Value=KOUTP_HVPwrSta_flg_ovrdflg
      link override Signal_Override/_ovrdval: Value=KOUTP_HVPwrSta_flg_ovrdval
  VPMM_HVSysReadyToCharge_enum_Inproc : FVT_lib/outp/OverrideAndLimit  SystemSampleTime=-1  VariantActivationTime=update diagram  Latency=0  AutoFrameSizeCalculation=off
      link override Signal_Limit/_maxval: Value=KOUTP_HVSysReadyToCharge_enum_maxval
      link override Signal_Limit/_minval: Value=KOUTP_HVSysReadyToCharge_enum_minval
      link override Signal_Override/_ovrdflg: Value=KOUTP_HVSysReadyToCharge_enum_ovrdflg
      link override Signal_Override/_ovrdval: Value=KOUTP_HVSysReadyToCharge_enum_ovrdval
  VPMM_HWResetSta_enum_Inproc : FVT_lib/outp/OverrideAndLimit  SystemSampleTime=-1  VariantActivationTime=update diagram  Latency=0  AutoFrameSizeCalculation=off
      link override Signal_Limit/_maxval: Value=KOUTP_HWResetSta_enum_maxval
      link override Signal_Limit/_minval: Value=KOUTP_HWResetSta_enum_minval
      link override Signal_Override/_ovrdflg: Value=KOUTP_HWResetSta_enum_ovrdflg
      link override Signal_Override/_ovrdval: Value=KOUTP_HWResetSta_enum_ovrdval
  VPMM_IVIPwrStaONTOPopT_s_Inproc : FVT_lib/outp/OverrideAndLimit  SystemSampleTime=-1  VariantActivationTime=update diagram  Latency=0  AutoFrameSizeCalculation=off
      link override Signal_Limit/_maxval: Value=KOUTP_IVIPwrStaONTOPopT_s_maxval
      link override Signal_Limit/_minval: Value=KOUTP_IVIPwrStaONTOPopT_s_minval
      link override Signal_Override/_ovrdflg: Value=KOUTP_IVIPwrStaONTOPopT_s_ovrdflg
      link override Signal_Override/_ovrdval: Value=KOUTP_IVIPwrStaONTOPopT_s_ovrdval
  VPMM_LVBattChrgTimeCnt_s_Inproc : FVT_lib/outp/OverrideAndLimit  SystemSampleTime=-1  VariantActivationTime=update diagram  Latency=0  AutoFrameSizeCalculation=off
      link override Signal_Limit/_maxval: Value=KOUTP_LVBattChrgTimeCnt_s_maxval
      link override Signal_Limit/_minval: Value=KOUTP_LVBattChrgTimeCnt_s_minval
      link override Signal_Override/_ovrdflg: Value=KOUTP_LVBattChrgTimeCnt_s_ovrdflg
      link override Signal_Override/_ovrdval: Value=KOUTP_LVBattChrgTimeCnt_s_ovrdval
  VPMM_LVChrgHoldTtimer_s_Inproc : FVT_lib/outp/OverrideAndLimit  SystemSampleTime=-1  VariantActivationTime=update diagram  Latency=0  AutoFrameSizeCalculation=off
      link override Signal_Limit/_maxval: Value=KOUTP_LVChrgHoldTtimer_s_maxval
      link override Signal_Limit/_minval: Value=KOUTP_LVChrgHoldTtimer_s_minval
      link override Signal_Override/_ovrdflg: Value=KOUTP_LVChrgHoldTtimer_s_ovrdflg
      link override Signal_Override/_ovrdval: Value=KOUTP_LVChrgHoldTtimer_s_ovrdval
  VPMM_LVPwrSta_flg_Inproc : FVT_lib/outp/OverrideAndLimit  SystemSampleTime=-1  VariantActivationTime=update diagram  Latency=0  AutoFrameSizeCalculation=off
      link override Signal_Limit/_maxval: Value=KOUTP_LVPwrSta_flg_maxval
      link override Signal_Limit/_minval: Value=KOUTP_LVPwrSta_flg_minval
      link override Signal_Override/_ovrdflg: Value=KOUTP_LVPwrSta_flg_ovrdflg
      link override Signal_Override/_ovrdval: Value=KOUTP_LVPwrSta_flg_ovrdval
  VPMM_LVSilentChrgLv_enum_Inproc : FVT_lib/outp/OverrideAndLimit  SystemSampleTime=-1  VariantActivationTime=update diagram  Latency=0  AutoFrameSizeCalculation=off
      link override Signal_Limit/_maxval: Value=KOUTP_LVSilentChrgLv_enum_maxval
      link override Signal_Limit/_minval: Value=KOUTP_LVSilentChrgLv_enum_minval
      link override Signal_Override/_ovrdflg: Value=KOUTP_LVSilentChrgLv_enum_ovrdflg
      link override Signal_Override/_ovrdval: Value=KOUTP_LVSilentChrgLv_enum_ovrdval
  VPMM_LVSilentChrgReq_flg_Inproc : FVT_lib/outp/OverrideAndLimit  SystemSampleTime=-1  VariantActivationTime=update diagram  Latency=0  AutoFrameSizeCalculation=off
      link override Signal_Limit/_maxval: Value=KOUTP_LVSilentChrgReq_flg_maxval
      link override Signal_Limit/_minval: Value=KOUTP_LVSilentChrgReq_flg_minval
      link override Signal_Override/_ovrdflg: Value=KOUTP_LVSilentChrgReq_flg_ovrdflg
      link override Signal_Override/_ovrdval: Value=KOUTP_LVSilentChrgReq_flg_ovrdval
  VPMM_LVSilentChrgSta_enum_Inproc : FVT_lib/outp/OverrideAndLimit  SystemSampleTime=-1  VariantActivationTime=update diagram  Latency=0  AutoFrameSizeCalculation=off
      link override Signal_Limit/_maxval: Value=KOUTP_LVSilentChrgSta_enum_maxval
      link override Signal_Limit/_minval: Value=KOUTP_LVSilentChrgSta_enum_minval
      link override Signal_Override/_ovrdflg: Value=KOUTP_LVSilentChrgSta_enum_ovrdflg
      link override Signal_Override/_ovrdval: Value=KOUTP_LVSilentChrgSta_enum_ovrdval
  VPMM_LVSysErrPwrOutErr_flg_Inproc : FVT_lib/outp/OverrideAndLimit  SystemSampleTime=-1  VariantActivationTime=update diagram  Latency=0  AutoFrameSizeCalculation=off
      link override Signal_Limit/_maxval: Value=KOUTP_LVSysErrPwrOutErr_flg_maxval
      link override Signal_Limit/_minval: Value=KOUTP_LVSysErrPwrOutErr_flg_minval
      link override Signal_Override/_ovrdflg: Value=KOUTP_LVSysErrPwrOutErr_flg_ovrdflg
      link override Signal_Override/_ovrdval: Value=KOUTP_LVSysErrPwrOutErr_flg_ovrdval
  VPMM_LowSOCWarn_enum_Inproc : FVT_lib/outp/OverrideAndLimit  SystemSampleTime=-1  VariantActivationTime=update diagram  Latency=0  AutoFrameSizeCalculation=off
      link override Signal_Limit/_maxval: Value=KOUTP_LowSOCWarn_enum_maxval
      link override Signal_Limit/_minval: Value=KOUTP_LowSOCWarn_enum_minval
      link override Signal_Override/_ovrdflg: Value=KOUTP_LowSOCWarn_enum_ovrdflg
      link override Signal_Override/_ovrdval: Value=KOUTP_LowSOCWarn_enum_ovrdval
  VPMM_OTAPwrReqOFFChkSta_enum_Inproc : FVT_lib/outp/OverrideAndLimit  SystemSampleTime=-1  VariantActivationTime=update diagram  Latency=0  AutoFrameSizeCalculation=off
      link override Signal_Limit/_maxval: Value=KOUTP_OTAPwrReqOFFChkSta_enum_maxval
      link override Signal_Limit/_minval: Value=KOUTP_OTAPwrReqOFFChkSta_enum_minval
      link override Signal_Override/_ovrdflg: Value=KOUTP_OTAPwrReqOFFChkSta_enum_ovrdflg
      link override Signal_Override/_ovrdval: Value=KOUTP_OTAPwrReqOFFChkSta_enum_ovrdval
  VPMM_OTAPwrReqStdChkSta_enum_Inproc : FVT_lib/outp/OverrideAndLimit  SystemSampleTime=-1  VariantActivationTime=update diagram  Latency=0  AutoFrameSizeCalculation=off
      link override Signal_Limit/_maxval: Value=KOUTP_OTAPwrReqStdChkSta_enum_maxval
      link override Signal_Limit/_minval: Value=KOUTP_OTAPwrReqStdChkSta_enum_minval
      link override Signal_Override/_ovrdflg: Value=KOUTP_OTAPwrReqStdChkSta_enum_ovrdflg
      link override Signal_Override/_ovrdval: Value=KOUTP_OTAPwrReqStdChkSta_enum_ovrdval
  VPMM_PMMAllowECUSleep_flg_Inproc : FVT_lib/outp/OverrideAndLimit  SystemSampleTime=-1  VariantActivationTime=update diagram  Latency=0  AutoFrameSizeCalculation=off
      link override Signal_Limit/_maxval: Value=KOUTP_PMMAllowECUSleep_flg_maxval
      link override Signal_Limit/_minval: Value=KOUTP_PMMAllowECUSleep_flg_minval
      link override Signal_Override/_ovrdflg: Value=KOUTP_PMMAllowECUSleep_flg_ovrdflg
      link override Signal_Override/_ovrdval: Value=KOUTP_PMMAllowECUSleep_flg_ovrdval
  VPMM_PowerDownFault_enum_Inproc : FVT_lib/outp/OverrideAndLimit  SystemSampleTime=-1  VariantActivationTime=update diagram  Latency=0  AutoFrameSizeCalculation=off
      link override Signal_Limit/_maxval: Value=KOUTP_PowerDownFault_enum_maxval
      link override Signal_Limit/_minval: Value=KOUTP_PowerDownFault_enum_minval
      link override Signal_Override/_ovrdflg: Value=KOUTP_PowerDownFault_enum_ovrdflg
      link override Signal_Override/_ovrdval: Value=KOUTP_PowerDownFault_enum_ovrdval
  VPMM_PowerDownState_enum_Inproc : FVT_lib/outp/OverrideAndLimit  SystemSampleTime=-1  VariantActivationTime=update diagram  Latency=0  AutoFrameSizeCalculation=off
      link override Signal_Limit/_maxval: Value=KOUTP_PowerDownState_enum_maxval
      link override Signal_Limit/_minval: Value=KOUTP_PowerDownState_enum_minval
      link override Signal_Override/_ovrdflg: Value=KOUTP_PowerDownState_enum_ovrdflg
      link override Signal_Override/_ovrdval: Value=KOUTP_PowerDownState_enum_ovrdval
  VPMM_PowerSta_enum_Inproc : FVT_lib/outp/OverrideAndLimit  SystemSampleTime=-1  VariantActivationTime=update diagram  Latency=0  AutoFrameSizeCalculation=off
      link override Signal_Limit/_maxval: Value=KOUTP_PowerSta_enum_maxval
      link override Signal_Limit/_minval: Value=KOUTP_PowerSta_enum_minval
      link override Signal_Override/_ovrdflg: Value=KOUTP_PowerSta_enum_ovrdflg
      link override Signal_Override/_ovrdval: Value=KOUTP_PowerSta_enum_ovrdval
  VPMM_PowerUpFault_enum_Inproc : FVT_lib/outp/OverrideAndLimit  SystemSampleTime=-1  VariantActivationTime=update diagram  Latency=0  AutoFrameSizeCalculation=off
      link override Signal_Limit/_maxval: Value=KOUTP_PowerUpFault_enum_maxval
      link override Signal_Limit/_minval: Value=KOUTP_PowerUpFault_enum_minval
      link override Signal_Override/_ovrdflg: Value=KOUTP_PowerUpFault_enum_ovrdflg
      link override Signal_Override/_ovrdval: Value=KOUTP_PowerUpFault_enum_ovrdval
  VPMM_PowerUpState_enum_Inproc : FVT_lib/outp/OverrideAndLimit  SystemSampleTime=-1  VariantActivationTime=update diagram  Latency=0  AutoFrameSizeCalculation=off
      link override Signal_Limit/_maxval: Value=KOUTP_PowerUpState_enum_maxval
      link override Signal_Limit/_minval: Value=KOUTP_PowerUpState_enum_minval
      link override Signal_Override/_ovrdflg: Value=KOUTP_PowerUpState_enum_ovrdflg
      link override Signal_Override/_ovrdval: Value=KOUTP_PowerUpState_enum_ovrdval
  VPMM_PwrDownReq_enum_Inproc : FVT_lib/outp/OverrideAndLimit  SystemSampleTime=-1  VariantActivationTime=update diagram  Latency=0  AutoFrameSizeCalculation=off
      link override Signal_Limit/_maxval: Value=KOUTP_PwrDownReq_enum_maxval
      link override Signal_Limit/_minval: Value=KOUTP_PwrDownReq_enum_minval
      link override Signal_Override/_ovrdflg: Value=KOUTP_PwrDownReq_enum_ovrdflg
      link override Signal_Override/_ovrdval: Value=KOUTP_PwrDownReq_enum_ovrdval
  VPMM_PwrReq_OTA_enum_Inproc : FVT_lib/outp/OverrideAndLimit  SystemSampleTime=-1  VariantActivationTime=update diagram  Latency=0  AutoFrameSizeCalculation=off
      link override Signal_Limit/_maxval: Value=KOUTP_PwrReq_OTA_enum_maxval
      link override Signal_Limit/_minval: Value=KOUTP_PwrReq_OTA_enum_minval
      link override Signal_Override/_ovrdflg: Value=KOUTP_PwrReq_OTA_enum_ovrdflg
      link override Signal_Override/_ovrdval: Value=KOUTP_PwrReq_OTA_enum_ovrdval
  VPMM_PwrStaConstraint_enum_Inproc : FVT_lib/outp/OverrideAndLimit  SystemSampleTime=-1  VariantActivationTime=update diagram  Latency=0  AutoFrameSizeCalculation=off
      link override Signal_Limit/_maxval: Value=KOUTP_PwrStaConstraint_enum_maxval
      link override Signal_Limit/_minval: Value=KOUTP_PwrStaConstraint_enum_minval
      link override Signal_Override/_ovrdflg: Value=KOUTP_PwrStaConstraint_enum_ovrdflg
      link override Signal_Override/_ovrdval: Value=KOUTP_PwrStaConstraint_enum_ovrdval
  VPMM_PwrStaONTOPopReq_flg_Inproc : FVT_lib/outp/OverrideAndLimit  SystemSampleTime=-1  VariantActivationTime=update diagram  Latency=0  AutoFrameSizeCalculation=off
      link override Signal_Limit/_maxval: Value=KOUTP_PwrStaONTOPopReq_flg_maxval
      link override Signal_Limit/_minval: Value=KOUTP_PwrStaONTOPopReq_flg_minval
      link override Signal_Override/_ovrdflg: Value=KOUTP_PwrStaONTOPopReq_flg_ovrdflg
      link override Signal_Override/_ovrdval: Value=KOUTP_PwrStaONTOPopReq_flg_ovrdval
  VPMM_PwrStaSelect_enum_Inproc : FVT_lib/outp/OverrideAndLimit  SystemSampleTime=-1  VariantActivationTime=update diagram  Latency=0  AutoFrameSizeCalculation=off
      link override Signal_Limit/_maxval: Value=KOUTP_PwrStaSelect_enum_maxval
      link override Signal_Limit/_minval: Value=KOUTP_PwrStaSelect_enum_minval
      link override Signal_Override/_ovrdflg: Value=KOUTP_PwrStaSelect_enum_ovrdflg
      link override Signal_Override/_ovrdval: Value=KOUTP_PwrStaSelect_enum_ovrdval
  VPMM_PwrStaTOSta_enum_Inproc : FVT_lib/outp/OverrideAndLimit  SystemSampleTime=-1  VariantActivationTime=update diagram  Latency=0  AutoFrameSizeCalculation=off
      link override Signal_Limit/_maxval: Value=KOUTP_PwrStaTOSta_enum_maxval
      link override Signal_Limit/_minval: Value=KOUTP_PwrStaTOSta_enum_minval
      link override Signal_Override/_ovrdflg: Value=KOUTP_PwrStaTOSta_enum_ovrdflg
      link override Signal_Override/_ovrdval: Value=KOUTP_PwrStaTOSta_enum_ovrdval
  VPMM_PwrUpReq_enum_Inproc : FVT_lib/outp/OverrideAndLimit  SystemSampleTime=-1  VariantActivationTime=update diagram  Latency=0  AutoFrameSizeCalculation=off
      link override Signal_Limit/_maxval: Value=KOUTP_PwrUpReq_enum_maxval
      link override Signal_Limit/_minval: Value=KOUTP_PwrUpReq_enum_minval
      link override Signal_Override/_ovrdflg: Value=KOUTP_PwrUpReq_enum_ovrdflg
      link override Signal_Override/_ovrdval: Value=KOUTP_PwrUpReq_enum_ovrdval
  VPMM_ReVehThdChkSta_enum_Inproc : FVT_lib/outp/OverrideAndLimit  SystemSampleTime=-1  VariantActivationTime=update diagram  Latency=0  AutoFrameSizeCalculation=off
      link override Signal_Limit/_maxval: Value=KOUTP_ReVehThdChkSta_enum_maxval
      link override Signal_Limit/_minval: Value=KOUTP_ReVehThdChkSta_enum_minval
      link override Signal_Override/_ovrdflg: Value=KOUTP_ReVehThdChkSta_enum_ovrdflg
      link override Signal_Override/_ovrdval: Value=KOUTP_ReVehThdChkSta_enum_ovrdval
  VPMM_RrMCUEnaReq_flg_Inproc : FVT_lib/outp/OverrideAndLimit  SystemSampleTime=-1  VariantActivationTime=update diagram  Latency=0  AutoFrameSizeCalculation=off
      link override Signal_Limit/_maxval: Value=KOUTP_RrMCUEnaReq_flg_maxval
      link override Signal_Limit/_minval: Value=KOUTP_RrMCUEnaReq_flg_minval
      link override Signal_Override/_ovrdflg: Value=KOUTP_RrMCUEnaReq_flg_ovrdflg
      link override Signal_Override/_ovrdval: Value=KOUTP_RrMCUEnaReq_flg_ovrdval
  VPMM_Sched_ChgTOSta_enum_Inproc : FVT_lib/outp/OverrideAndLimit  SystemSampleTime=-1  VariantActivationTime=update diagram  Latency=0  AutoFrameSizeCalculation=off
      link override Signal_Limit/_maxval: Value=KOUTP_Sched_ChgTOSta_enum_maxval
      link override Signal_Limit/_minval: Value=KOUTP_Sched_ChgTOSta_enum_minval
      link override Signal_Override/_ovrdflg: Value=KOUTP_Sched_ChgTOSta_enum_ovrdflg
      link override Signal_Override/_ovrdval: Value=KOUTP_Sched_ChgTOSta_enum_ovrdval
  VPMM_SilentChkAllowSleep_flg_Inproc : FVT_lib/outp/OverrideAndLimit  SystemSampleTime=-1  VariantActivationTime=update diagram  Latency=0  AutoFrameSizeCalculation=off
      link override Signal_Limit/_maxval: Value=KOUTP_SilentChkAllowSleep_flg_maxval
      link override Signal_Limit/_minval: Value=KOUTP_SilentChkAllowSleep_flg_minval
      link override Signal_Override/_ovrdflg: Value=KOUTP_SilentChkAllowSleep_flg_ovrdflg
      link override Signal_Override/_ovrdval: Value=KOUTP_SilentChkAllowSleep_flg_ovrdval
  VPMM_SysPowerMode_enum_Inproc : FVT_lib/outp/OverrideAndLimit  SystemSampleTime=-1  VariantActivationTime=update diagram  Latency=0  AutoFrameSizeCalculation=off
      link override Signal_Limit/_maxval: Value=KOUTP_SysPowerMode_enum_maxval
      link override Signal_Limit/_minval: Value=KOUTP_SysPowerMode_enum_minval
      link override Signal_Override/_ovrdflg: Value=KOUTP_SysPowerMode_enum_ovrdflg
      link override Signal_Override/_ovrdval: Value=KOUTP_SysPowerMode_enum_ovrdval
  VPMM_TCountSta_enum_Inproc : FVT_lib/outp/OverrideAndLimit  SystemSampleTime=-1  VariantActivationTime=update diagram  Latency=0  AutoFrameSizeCalculation=off
      link override Signal_Limit/_maxval: Value=KOUTP_TCountSta_enum_maxval
      link override Signal_Limit/_minval: Value=KOUTP_TCountSta_enum_minval
      link override Signal_Override/_ovrdflg: Value=KOUTP_TCountSta_enum_ovrdflg
      link override Signal_Override/_ovrdval: Value=KOUTP_TCountSta_enum_ovrdval
  VPMM_TimerAllowSleep_flg_Inproc : FVT_lib/outp/OverrideAndLimit  SystemSampleTime=-1  VariantActivationTime=update diagram  Latency=0  AutoFrameSizeCalculation=off
      link override Signal_Limit/_maxval: Value=KOUTP_TimerAllowSleep_flg_maxval
      link override Signal_Limit/_minval: Value=KOUTP_TimerAllowSleep_flg_minval
      link override Signal_Override/_ovrdflg: Value=KOUTP_TimerAllowSleep_flg_ovrdflg
      link override Signal_Override/_ovrdval: Value=KOUTP_TimerAllowSleep_flg_ovrdval
  VSYS_AcoreRebootCmdACK_flg_Inproc : FVT_lib/outp/OverrideAndLimit  SystemSampleTime=-1  VariantActivationTime=update diagram  Latency=0  AutoFrameSizeCalculation=off
      link override Signal_Limit/_maxval: Value=KOUTP_AcoreRebootCmdACK_flg_maxval
      link override Signal_Limit/_minval: Value=KOUTP_AcoreRebootCmdACK_flg_minval
      link override Signal_Override/_ovrdflg: Value=KOUTP_AcoreRebootCmdACK_flg_ovrdflg
      link override Signal_Override/_ovrdval: Value=KOUTP_AcoreRebootCmdACK_flg_ovrdval
  VSYS_CarModel1_cnt_Inproc : FVT_lib/outp/OverrideAndLimit  SystemSampleTime=-1  VariantActivationTime=update diagram  Latency=0  AutoFrameSizeCalculation=off
      link override Signal_Limit/_maxval: Value=KOUTP_CarModel1_cnt_maxval
      link override Signal_Limit/_minval: Value=KOUTP_CarModel1_cnt_minval
      link override Signal_Override/_ovrdflg: Value=KOUTP_CarModel1_cnt_ovrdflg
      link override Signal_Override/_ovrdval: Value=KOUTP_CarModel1_cnt_ovrdval
  VSYS_CarModel2_cnt_Inproc : FVT_lib/outp/OverrideAndLimit  SystemSampleTime=-1  VariantActivationTime=update diagram  Latency=0  AutoFrameSizeCalculation=off
      link override Signal_Limit/_maxval: Value=KOUTP_CarModel2_cnt_maxval
      link override Signal_Limit/_minval: Value=KOUTP_CarModel2_cnt_minval
      link override Signal_Override/_ovrdflg: Value=KOUTP_CarModel2_cnt_ovrdflg
      link override Signal_Override/_ovrdval: Value=KOUTP_CarModel2_cnt_ovrdval
  VSYS_CarModel3_cnt_Inproc : FVT_lib/outp/OverrideAndLimit  SystemSampleTime=-1  VariantActivationTime=update diagram  Latency=0  AutoFrameSizeCalculation=off
      link override Signal_Limit/_maxval: Value=KOUTP_CarModel3_cnt_maxval
      link override Signal_Limit/_minval: Value=KOUTP_CarModel3_cnt_minval
      link override Signal_Override/_ovrdflg: Value=KOUTP_CarModel3_cnt_ovrdflg
      link override Signal_Override/_ovrdval: Value=KOUTP_CarModel3_cnt_ovrdval
  VSYS_Change1_cnt_Inproc : FVT_lib/outp/OverrideAndLimit  SystemSampleTime=-1  VariantActivationTime=update diagram  Latency=0  AutoFrameSizeCalculation=off
      link override Signal_Limit/_maxval: Value=KOUTP_Change1_cnt_maxval
      link override Signal_Limit/_minval: Value=KOUTP_Change1_cnt_minval
      link override Signal_Override/_ovrdflg: Value=KOUTP_Change1_cnt_ovrdflg
      link override Signal_Override/_ovrdval: Value=KOUTP_Change1_cnt_ovrdval
  VSYS_Change2_cnt_Inproc : FVT_lib/outp/OverrideAndLimit  SystemSampleTime=-1  VariantActivationTime=update diagram  Latency=0  AutoFrameSizeCalculation=off
      link override Signal_Limit/_maxval: Value=KOUTP_Change2_cnt_maxval
      link override Signal_Limit/_minval: Value=KOUTP_Change2_cnt_minval
      link override Signal_Override/_ovrdflg: Value=KOUTP_Change2_cnt_ovrdflg
      link override Signal_Override/_ovrdval: Value=KOUTP_Change2_cnt_ovrdval
  VSYS_Country1_cnt_Inproc : FVT_lib/outp/OverrideAndLimit  SystemSampleTime=-1  VariantActivationTime=update diagram  Latency=0  AutoFrameSizeCalculation=off
      link override Signal_Limit/_maxval: Value=KOUTP_Country1_cnt_maxval
      link override Signal_Limit/_minval: Value=KOUTP_Country1_cnt_minval
      link override Signal_Override/_ovrdflg: Value=KOUTP_Country1_cnt_ovrdflg
      link override Signal_Override/_ovrdval: Value=KOUTP_Country1_cnt_ovrdval
  VSYS_Country2_cnt_Inproc : FVT_lib/outp/OverrideAndLimit  SystemSampleTime=-1  VariantActivationTime=update diagram  Latency=0  AutoFrameSizeCalculation=off
      link override Signal_Limit/_maxval: Value=KOUTP_Country2_cnt_maxval
      link override Signal_Limit/_minval: Value=KOUTP_Country2_cnt_minval
      link override Signal_Override/_ovrdflg: Value=KOUTP_Country2_cnt_ovrdflg
      link override Signal_Override/_ovrdval: Value=KOUTP_Country2_cnt_ovrdval
  VSYS_CurrentNmState_enum_Inproc : FVT_lib/outp/OverrideAndLimit  SystemSampleTime=-1  VariantActivationTime=update diagram  Latency=0  AutoFrameSizeCalculation=off
      link override Signal_Limit/_maxval: Value=KOUTP_CurrentNmState_enum_maxval
      link override Signal_Limit/_minval: Value=KOUTP_CurrentNmState_enum_minval
      link override Signal_Override/_ovrdflg: Value=KOUTP_CurrentNmState_enum_ovrdflg
      link override Signal_Override/_ovrdval: Value=KOUTP_CurrentNmState_enum_ovrdval
  VSYS_Dash1_cnt_Inproc : FVT_lib/outp/OverrideAndLimit  SystemSampleTime=-1  VariantActivationTime=update diagram  Latency=0  AutoFrameSizeCalculation=off
      link override Signal_Limit/_maxval: Value=KOUTP_Dash1_cnt_maxval
      link override Signal_Limit/_minval: Value=KOUTP_Dash1_cnt_minval
      link override Signal_Override/_ovrdflg: Value=KOUTP_Dash1_cnt_ovrdflg
      link override Signal_Override/_ovrdval: Value=KOUTP_Dash1_cnt_ovrdval
  VSYS_Dash2_cnt_Inproc : FVT_lib/outp/OverrideAndLimit  SystemSampleTime=-1  VariantActivationTime=update diagram  Latency=0  AutoFrameSizeCalculation=off
      link override Signal_Limit/_maxval: Value=KOUTP_Dash2_cnt_maxval
      link override Signal_Limit/_minval: Value=KOUTP_Dash2_cnt_minval
      link override Signal_Override/_ovrdflg: Value=KOUTP_Dash2_cnt_ovrdflg
      link override Signal_Override/_ovrdval: Value=KOUTP_Dash2_cnt_ovrdval
  VSYS_ECU1_cnt_Inproc : FVT_lib/outp/OverrideAndLimit  SystemSampleTime=-1  VariantActivationTime=update diagram  Latency=0  AutoFrameSizeCalculation=off
      link override Signal_Limit/_maxval: Value=KOUTP_ECU1_cnt_maxval
      link override Signal_Limit/_minval: Value=KOUTP_ECU1_cnt_minval
      link override Signal_Override/_ovrdflg: Value=KOUTP_ECU1_cnt_ovrdflg
      link override Signal_Override/_ovrdval: Value=KOUTP_ECU1_cnt_ovrdval
  VSYS_ECU2_cnt_Inproc : FVT_lib/outp/OverrideAndLimit  SystemSampleTime=-1  VariantActivationTime=update diagram  Latency=0  AutoFrameSizeCalculation=off
      link override Signal_Limit/_maxval: Value=KOUTP_ECU2_cnt_maxval
      link override Signal_Limit/_minval: Value=KOUTP_ECU2_cnt_minval
      link override Signal_Override/_ovrdflg: Value=KOUTP_ECU2_cnt_ovrdflg
      link override Signal_Override/_ovrdval: Value=KOUTP_ECU2_cnt_ovrdval
  VSYS_FdcSlpReqRisingEdge_flg_Inproc : FVT_lib/outp/OverrideAndLimit  SystemSampleTime=-1  VariantActivationTime=update diagram  Latency=0  AutoFrameSizeCalculation=off
      link override Signal_Limit/_maxval: Value=KOUTP_FdcSlpReqRisingEdge_flg_maxval
      link override Signal_Limit/_minval: Value=KOUTP_FdcSlpReqRisingEdge_flg_minval
      link override Signal_Override/_ovrdflg: Value=KOUTP_FdcSlpReqRisingEdge_flg_ovrdflg
      link override Signal_Override/_ovrdval: Value=KOUTP_FdcSlpReqRisingEdge_flg_ovrdval
  VSYS_FdcSlpTime_sec_Inproc : FVT_lib/outp/OverrideAndLimit  SystemSampleTime=-1  VariantActivationTime=update diagram  Latency=0  AutoFrameSizeCalculation=off
      link override Signal_Limit/_maxval: Value=KOUTP_FdcSlpTime_sec_maxval
      link override Signal_Limit/_minval: Value=KOUTP_FdcSlpTime_sec_minval
      link override Signal_Override/_ovrdflg: Value=KOUTP_FdcSlpTime_sec_ovrdflg
      link override Signal_Override/_ovrdval: Value=KOUTP_FdcSlpTime_sec_ovrdval
  VSYS_HWVer1_cnt_Inproc : FVT_lib/outp/OverrideAndLimit  SystemSampleTime=-1  VariantActivationTime=update diagram  Latency=0  AutoFrameSizeCalculation=off
      link override Signal_Limit/_maxval: Value=KOUTP_HWVer1_cnt_maxval
      link override Signal_Limit/_minval: Value=KOUTP_HWVer1_cnt_minval
      link override Signal_Override/_ovrdflg: Value=KOUTP_HWVer1_cnt_ovrdflg
      link override Signal_Override/_ovrdval: Value=KOUTP_HWVer1_cnt_ovrdval
  VSYS_HWVer2_cnt_Inproc : FVT_lib/outp/OverrideAndLimit  SystemSampleTime=-1  VariantActivationTime=update diagram  Latency=0  AutoFrameSizeCalculation=off
      link override Signal_Limit/_maxval: Value=KOUTP_HWVer2_cnt_maxval
      link override Signal_Limit/_minval: Value=KOUTP_HWVer2_cnt_minval
      link override Signal_Override/_ovrdflg: Value=KOUTP_HWVer2_cnt_ovrdflg
      link override Signal_Override/_ovrdval: Value=KOUTP_HWVer2_cnt_ovrdval
  VSYS_HWVer3_cnt_Inproc : FVT_lib/outp/OverrideAndLimit  SystemSampleTime=-1  VariantActivationTime=update diagram  Latency=0  AutoFrameSizeCalculation=off
      link override Signal_Limit/_maxval: Value=KOUTP_HWVer3_cnt_maxval
      link override Signal_Limit/_minval: Value=KOUTP_HWVer3_cnt_minval
      link override Signal_Override/_ovrdflg: Value=KOUTP_HWVer3_cnt_ovrdflg
      link override Signal_Override/_ovrdval: Value=KOUTP_HWVer3_cnt_ovrdval
  VSYS_Major1_cnt_Inproc : FVT_lib/outp/OverrideAndLimit  SystemSampleTime=-1  VariantActivationTime=update diagram  Latency=0  AutoFrameSizeCalculation=off
      link override Signal_Limit/_maxval: Value=KOUTP_Major1_cnt_maxval
      link override Signal_Limit/_minval: Value=KOUTP_Major1_cnt_minval
      link override Signal_Override/_ovrdflg: Value=KOUTP_Major1_cnt_ovrdflg
      link override Signal_Override/_ovrdval: Value=KOUTP_Major1_cnt_ovrdval
  VSYS_Major2_cnt_Inproc : FVT_lib/outp/OverrideAndLimit  SystemSampleTime=-1  VariantActivationTime=update diagram  Latency=0  AutoFrameSizeCalculation=off
      link override Signal_Limit/_maxval: Value=KOUTP_Major2_cnt_maxval
      link override Signal_Limit/_minval: Value=KOUTP_Major2_cnt_minval
      link override Signal_Override/_ovrdflg: Value=KOUTP_Major2_cnt_ovrdflg
      link override Signal_Override/_ovrdval: Value=KOUTP_Major2_cnt_ovrdval
  VSYS_Minor1_cnt_Inproc : FVT_lib/outp/OverrideAndLimit  SystemSampleTime=-1  VariantActivationTime=update diagram  Latency=0  AutoFrameSizeCalculation=off
      link override Signal_Limit/_maxval: Value=KOUTP_Minor1_cnt_maxval
      link override Signal_Limit/_minval: Value=KOUTP_Minor1_cnt_minval
      link override Signal_Override/_ovrdflg: Value=KOUTP_Minor1_cnt_ovrdflg
      link override Signal_Override/_ovrdval: Value=KOUTP_Minor1_cnt_ovrdval
  VSYS_Minor2_cnt_Inproc : FVT_lib/outp/OverrideAndLimit  SystemSampleTime=-1  VariantActivationTime=update diagram  Latency=0  AutoFrameSizeCalculation=off
      link override Signal_Limit/_maxval: Value=KOUTP_Minor2_cnt_maxval
      link override Signal_Limit/_minval: Value=KOUTP_Minor2_cnt_minval
      link override Signal_Override/_ovrdflg: Value=KOUTP_Minor2_cnt_ovrdflg
      link override Signal_Override/_ovrdval: Value=KOUTP_Minor2_cnt_ovrdval
  VSYS_NvWriteReqRisingEdge_flg_Inproc : FVT_lib/outp/OverrideAndLimit  SystemSampleTime=-1  VariantActivationTime=update diagram  Latency=0  AutoFrameSizeCalculation=off
      link override Signal_Limit/_maxval: Value=KOUTP_NvWriteReqRisingEdge_flg_maxval
      link override Signal_Limit/_minval: Value=KOUTP_NvWriteReqRisingEdge_flg_minval
      link override Signal_Override/_ovrdflg: Value=KOUTP_NvWriteReqRisingEdge_flg_ovrdflg
      link override Signal_Override/_ovrdval: Value=KOUTP_NvWriteReqRisingEdge_flg_ovrdval
  VSYS_Patch1_cnt_Inproc : FVT_lib/outp/OverrideAndLimit  SystemSampleTime=-1  VariantActivationTime=update diagram  Latency=0  AutoFrameSizeCalculation=off
      link override Signal_Limit/_maxval: Value=KOUTP_Patch1_cnt_maxval
      link override Signal_Limit/_minval: Value=KOUTP_Patch1_cnt_minval
      link override Signal_Override/_ovrdflg: Value=KOUTP_Patch1_cnt_ovrdflg
      link override Signal_Override/_ovrdval: Value=KOUTP_Patch1_cnt_ovrdval
  VSYS_Patch2_cnt_Inproc : FVT_lib/outp/OverrideAndLimit  SystemSampleTime=-1  VariantActivationTime=update diagram  Latency=0  AutoFrameSizeCalculation=off
      link override Signal_Limit/_maxval: Value=KOUTP_Patch2_cnt_maxval
      link override Signal_Limit/_minval: Value=KOUTP_Patch2_cnt_minval
      link override Signal_Override/_ovrdflg: Value=KOUTP_Patch2_cnt_ovrdflg
      link override Signal_Override/_ovrdval: Value=KOUTP_Patch2_cnt_ovrdval
  VSYS_PmicBootReason_enum_Inproc : FVT_lib/outp/OverrideAndLimit  SystemSampleTime=-1  VariantActivationTime=update diagram  Latency=0  AutoFrameSizeCalculation=off
      link override Signal_Limit/_maxval: Value=KOUTP_PmicBootReason_enum_maxval
      link override Signal_Limit/_minval: Value=KOUTP_PmicBootReason_enum_minval
      link override Signal_Override/_ovrdflg: Value=KOUTP_PmicBootReason_enum_ovrdflg
      link override Signal_Override/_ovrdval: Value=KOUTP_PmicBootReason_enum_ovrdval
  VSYS_SHA1_cnt_Inproc : FVT_lib/outp/OverrideAndLimit  SystemSampleTime=-1  VariantActivationTime=update diagram  Latency=0  AutoFrameSizeCalculation=off
      link override Signal_Limit/_maxval: Value=KOUTP_SHA1_cnt_maxval
      link override Signal_Limit/_minval: Value=KOUTP_SHA1_cnt_minval
      link override Signal_Override/_ovrdflg: Value=KOUTP_SHA1_cnt_ovrdflg
      link override Signal_Override/_ovrdval: Value=KOUTP_SHA1_cnt_ovrdval
  VSYS_SHA2_cnt_Inproc : FVT_lib/outp/OverrideAndLimit  SystemSampleTime=-1  VariantActivationTime=update diagram  Latency=0  AutoFrameSizeCalculation=off
      link override Signal_Limit/_maxval: Value=KOUTP_SHA2_cnt_maxval
      link override Signal_Limit/_minval: Value=KOUTP_SHA2_cnt_minval
      link override Signal_Override/_ovrdflg: Value=KOUTP_SHA2_cnt_ovrdflg
      link override Signal_Override/_ovrdval: Value=KOUTP_SHA2_cnt_ovrdval
  VSYS_SHA3_cnt_Inproc : FVT_lib/outp/OverrideAndLimit  SystemSampleTime=-1  VariantActivationTime=update diagram  Latency=0  AutoFrameSizeCalculation=off
      link override Signal_Limit/_maxval: Value=KOUTP_SHA3_cnt_maxval
      link override Signal_Limit/_minval: Value=KOUTP_SHA3_cnt_minval
      link override Signal_Override/_ovrdflg: Value=KOUTP_SHA3_cnt_ovrdflg
      link override Signal_Override/_ovrdval: Value=KOUTP_SHA3_cnt_ovrdval
  VSYS_SHA4_cnt_Inproc : FVT_lib/outp/OverrideAndLimit  SystemSampleTime=-1  VariantActivationTime=update diagram  Latency=0  AutoFrameSizeCalculation=off
      link override Signal_Limit/_maxval: Value=KOUTP_SHA4_cnt_maxval
      link override Signal_Limit/_minval: Value=KOUTP_SHA4_cnt_minval
      link override Signal_Override/_ovrdflg: Value=KOUTP_SHA4_cnt_ovrdflg
      link override Signal_Override/_ovrdval: Value=KOUTP_SHA4_cnt_ovrdval
  VSYS_SHA5_cnt_Inproc : FVT_lib/outp/OverrideAndLimit  SystemSampleTime=-1  VariantActivationTime=update diagram  Latency=0  AutoFrameSizeCalculation=off
      link override Signal_Limit/_maxval: Value=KOUTP_SHA5_cnt_maxval
      link override Signal_Limit/_minval: Value=KOUTP_SHA5_cnt_minval
      link override Signal_Override/_ovrdflg: Value=KOUTP_SHA5_cnt_ovrdflg
      link override Signal_Override/_ovrdval: Value=KOUTP_SHA5_cnt_ovrdval
  VSYS_SHA6_cnt_Inproc : FVT_lib/outp/OverrideAndLimit  SystemSampleTime=-1  VariantActivationTime=update diagram  Latency=0  AutoFrameSizeCalculation=off
      link override Signal_Limit/_maxval: Value=KOUTP_SHA6_cnt_maxval
      link override Signal_Limit/_minval: Value=KOUTP_SHA6_cnt_minval
      link override Signal_Override/_ovrdflg: Value=KOUTP_SHA6_cnt_ovrdflg
      link override Signal_Override/_ovrdval: Value=KOUTP_SHA6_cnt_ovrdval
  VSYS_SHA7_cnt_Inproc : FVT_lib/outp/OverrideAndLimit  SystemSampleTime=-1  VariantActivationTime=update diagram  Latency=0  AutoFrameSizeCalculation=off
      link override Signal_Limit/_maxval: Value=KOUTP_SHA7_cnt_maxval
      link override Signal_Limit/_minval: Value=KOUTP_SHA7_cnt_minval
      link override Signal_Override/_ovrdflg: Value=KOUTP_SHA7_cnt_ovrdflg
      link override Signal_Override/_ovrdval: Value=KOUTP_SHA7_cnt_ovrdval
  VSYS_SHA8_cnt_Inproc : FVT_lib/outp/OverrideAndLimit  SystemSampleTime=-1  VariantActivationTime=update diagram  Latency=0  AutoFrameSizeCalculation=off
      link override Signal_Limit/_maxval: Value=KOUTP_SHA8_cnt_maxval
      link override Signal_Limit/_minval: Value=KOUTP_SHA8_cnt_minval
      link override Signal_Override/_ovrdflg: Value=KOUTP_SHA8_cnt_ovrdflg
      link override Signal_Override/_ovrdval: Value=KOUTP_SHA8_cnt_ovrdval
  VSYS_Variation_cnt_Inproc : FVT_lib/outp/OverrideAndLimit  SystemSampleTime=-1  VariantActivationTime=update diagram  Latency=0  AutoFrameSizeCalculation=off
      link override Signal_Limit/_maxval: Value=KOUTP_Variation_cnt_maxval
      link override Signal_Limit/_minval: Value=KOUTP_Variation_cnt_minval
      link override Signal_Override/_ovrdflg: Value=KOUTP_Variation_cnt_ovrdflg
      link override Signal_Override/_ovrdval: Value=KOUTP_Variation_cnt_ovrdval
  VSYS_WisrBootReason_raw32_Inproc : FVT_lib/outp/OverrideAndLimit  SystemSampleTime=-1  VariantActivationTime=update diagram  Latency=0  AutoFrameSizeCalculation=off
      link override Signal_Limit/_maxval: Value=KOUTP_WisrBootReason_raw32_maxval
      link override Signal_Limit/_minval: Value=KOUTP_WisrBootReason_raw32_minval
      link override Signal_Override/_ovrdflg: Value=KOUTP_WisrBootReason_raw32_ovrdflg
      link override Signal_Override/_ovrdval: Value=KOUTP_WisrBootReason_raw32_ovrdval
  VTHC_ACForceOFF_flg_Inproc : FVT_lib/outp/OverrideAndLimit  SystemSampleTime=-1  VariantActivationTime=update diagram  Latency=0  AutoFrameSizeCalculation=off
      link override Signal_Limit/_maxval: Value=KOUTP_ACForceOFF_flg_maxval
      link override Signal_Limit/_minval: Value=KOUTP_ACForceOFF_flg_minval
      link override Signal_Override/_ovrdflg: Value=KOUTP_ACForceOFF_flg_ovrdflg
      link override Signal_Override/_ovrdval: Value=KOUTP_ACForceOFF_flg_ovrdval
  VTHC_ACModeMem_enum_Inproc : FVT_lib/outp/OverrideAndLimit  SystemSampleTime=-1  VariantActivationTime=update diagram  Latency=0  AutoFrameSizeCalculation=off
      link override Signal_Limit/_maxval: Value=KOUTP_ACModeMem_enum_maxval
      link override Signal_Limit/_minval: Value=KOUTP_ACModeMem_enum_minval
      link override Signal_Override/_ovrdflg: Value=KOUTP_ACModeMem_enum_ovrdflg
      link override Signal_Override/_ovrdval: Value=KOUTP_ACModeMem_enum_ovrdval
  VTHC_ACSubMode_enum_Inproc : FVT_lib/outp/OverrideAndLimit  SystemSampleTime=-1  VariantActivationTime=update diagram  Latency=0  AutoFrameSizeCalculation=off
      link override Signal_Limit/_maxval: Value=KOUTP_ACSubMode_enum_maxval
      link override Signal_Limit/_minval: Value=KOUTP_ACSubMode_enum_minval
      link override Signal_Override/_ovrdflg: Value=KOUTP_ACSubMode_enum_ovrdflg
      link override Signal_Override/_ovrdval: Value=KOUTP_ACSubMode_enum_ovrdval
  VTHC_AirIntenZone1M_enum_Inproc : FVT_lib/outp/OverrideAndLimit  SystemSampleTime=-1  VariantActivationTime=update diagram  Latency=0  AutoFrameSizeCalculation=off
      link override Signal_Limit/_maxval: Value=KOUTP_AirIntenZone1M_enum_maxval
      link override Signal_Limit/_minval: Value=KOUTP_AirIntenZone1M_enum_minval
      link override Signal_Override/_ovrdflg: Value=KOUTP_AirIntenZone1M_enum_ovrdflg
      link override Signal_Override/_ovrdval: Value=KOUTP_AirIntenZone1M_enum_ovrdval
  VTHC_BatteryMode_enum_Inproc : FVT_lib/outp/OverrideAndLimit  SystemSampleTime=-1  VariantActivationTime=update diagram  Latency=0  AutoFrameSizeCalculation=off
      link override Signal_Limit/_maxval: Value=KOUTP_BatteryMode_enum_maxval
      link override Signal_Limit/_minval: Value=KOUTP_BatteryMode_enum_minval
      link override Signal_Override/_ovrdflg: Value=KOUTP_BatteryMode_enum_ovrdflg
      link override Signal_Override/_ovrdval: Value=KOUTP_BatteryMode_enum_ovrdval
  VTHC_CCUACLampSts_flg_Inproc : FVT_lib/outp/OverrideAndLimit  SystemSampleTime=-1  VariantActivationTime=update diagram  Latency=0  AutoFrameSizeCalculation=off
      link override Signal_Limit/_maxval: Value=KOUTP_CCUACLampSts_flg_maxval
      link override Signal_Limit/_minval: Value=KOUTP_CCUACLampSts_flg_minval
      link override Signal_Override/_ovrdflg: Value=KOUTP_CCUACLampSts_flg_ovrdflg
      link override Signal_Override/_ovrdval: Value=KOUTP_CCUACLampSts_flg_ovrdval
  VTHC_CCUACMaxLampSts_flg_Inproc : FVT_lib/outp/OverrideAndLimit  SystemSampleTime=-1  VariantActivationTime=update diagram  Latency=0  AutoFrameSizeCalculation=off
      link override Signal_Limit/_maxval: Value=KOUTP_CCUACMaxLampSts_flg_maxval
      link override Signal_Limit/_minval: Value=KOUTP_CCUACMaxLampSts_flg_minval
      link override Signal_Override/_ovrdflg: Value=KOUTP_CCUACMaxLampSts_flg_ovrdflg
      link override Signal_Override/_ovrdval: Value=KOUTP_CCUACMaxLampSts_flg_ovrdval
  VTHC_CCUAutoLampSts_flg_Inproc : FVT_lib/outp/OverrideAndLimit  SystemSampleTime=-1  VariantActivationTime=update diagram  Latency=0  AutoFrameSizeCalculation=off
      link override Signal_Limit/_maxval: Value=KOUTP_CCUAutoLampSts_flg_maxval
      link override Signal_Limit/_minval: Value=KOUTP_CCUAutoLampSts_flg_minval
      link override Signal_Override/_ovrdflg: Value=KOUTP_CCUAutoLampSts_flg_ovrdflg
      link override Signal_Override/_ovrdval: Value=KOUTP_CCUAutoLampSts_flg_ovrdval
  VTHC_CCUSyncLampSts_flg_Inproc : FVT_lib/outp/OverrideAndLimit  SystemSampleTime=-1  VariantActivationTime=update diagram  Latency=0  AutoFrameSizeCalculation=off
      link override Signal_Limit/_maxval: Value=KOUTP_CCUSyncLampSts_flg_maxval
      link override Signal_Limit/_minval: Value=KOUTP_CCUSyncLampSts_flg_minval
      link override Signal_Override/_ovrdflg: Value=KOUTP_CCUSyncLampSts_flg_ovrdflg
      link override Signal_Override/_ovrdval: Value=KOUTP_CCUSyncLampSts_flg_ovrdval
  VTHC_CCUSyncSts_flg_Inproc : FVT_lib/outp/OverrideAndLimit  SystemSampleTime=-1  VariantActivationTime=update diagram  Latency=0  AutoFrameSizeCalculation=off
      link override Signal_Limit/_maxval: Value=KOUTP_CCUSyncSts_flg_maxval
      link override Signal_Limit/_minval: Value=KOUTP_CCUSyncSts_flg_minval
      link override Signal_Override/_ovrdflg: Value=KOUTP_CCUSyncSts_flg_ovrdflg
      link override Signal_Override/_ovrdval: Value=KOUTP_CCUSyncSts_flg_ovrdval
  VTHC_CabinMode_enum_Inproc : FVT_lib/outp/OverrideAndLimit  SystemSampleTime=-1  VariantActivationTime=update diagram  Latency=0  AutoFrameSizeCalculation=off
      link override Signal_Limit/_maxval: Value=KOUTP_CabinMode_enum_maxval
      link override Signal_Limit/_minval: Value=KOUTP_CabinMode_enum_minval
      link override Signal_Override/_ovrdflg: Value=KOUTP_CabinMode_enum_ovrdflg
      link override Signal_Override/_ovrdval: Value=KOUTP_CabinMode_enum_ovrdval
  VTHC_CoolgFanActDuty_pct_Inproc : FVT_lib/outp/OverrideAndLimit  SystemSampleTime=-1  VariantActivationTime=update diagram  Latency=0  AutoFrameSizeCalculation=off
      link override Signal_Limit/_maxval: Value=KOUTP_CoolgFanActDuty_pct_maxval
      link override Signal_Limit/_minval: Value=KOUTP_CoolgFanActDuty_pct_minval
      link override Signal_Override/_ovrdflg: Value=KOUTP_CoolgFanActDuty_pct_ovrdflg
      link override Signal_Override/_ovrdval: Value=KOUTP_CoolgFanActDuty_pct_ovrdval
  VTHC_EDriveMode_enum_Inproc : FVT_lib/outp/OverrideAndLimit  SystemSampleTime=-1  VariantActivationTime=update diagram  Latency=0  AutoFrameSizeCalculation=off
      link override Signal_Limit/_maxval: Value=KOUTP_EDriveMode_enum_maxval
      link override Signal_Limit/_minval: Value=KOUTP_EDriveMode_enum_minval
      link override Signal_Override/_ovrdflg: Value=KOUTP_EDriveMode_enum_ovrdflg
      link override Signal_Override/_ovrdval: Value=KOUTP_EDriveMode_enum_ovrdval
  VTHC_FDAGSCmd_enum_Inproc : FVT_lib/outp/OverrideAndLimit  SystemSampleTime=-1  VariantActivationTime=update diagram  Latency=0  AutoFrameSizeCalculation=off
      link override Signal_Limit/_maxval: Value=KOUTP_FDAGSCmd_enum_maxval
      link override Signal_Limit/_minval: Value=KOUTP_FDAGSCmd_enum_minval
      link override Signal_Override/_ovrdflg: Value=KOUTP_FDAGSCmd_enum_ovrdflg
      link override Signal_Override/_ovrdval: Value=KOUTP_FDAGSCmd_enum_ovrdval
  VTHC_FDBlowerCmd_pct_Inproc : FVT_lib/outp/OverrideAndLimit  SystemSampleTime=-1  VariantActivationTime=update diagram  Latency=0  AutoFrameSizeCalculation=off
      link override Signal_Limit/_maxval: Value=KOUTP_FDBlowerCmd_pct_maxval
      link override Signal_Limit/_minval: Value=KOUTP_FDBlowerCmd_pct_minval
      link override Signal_Override/_ovrdflg: Value=KOUTP_FDBlowerCmd_pct_ovrdflg
      link override Signal_Override/_ovrdval: Value=KOUTP_FDBlowerCmd_pct_ovrdval
  VTHC_FDCTHCMAPTCWarningSta_flg_Inproc : FVT_lib/outp/OverrideAndLimit  SystemSampleTime=-1  VariantActivationTime=update diagram  Latency=0  AutoFrameSizeCalculation=off
      link override Signal_Limit/_maxval: Value=KOUTP_FDCTHCMAPTCWarningSta_flg_maxval
      link override Signal_Limit/_minval: Value=KOUTP_FDCTHCMAPTCWarningSta_flg_minval
      link override Signal_Override/_ovrdflg: Value=KOUTP_FDCTHCMAPTCWarningSta_flg_ovrdflg
      link override Signal_Override/_ovrdval: Value=KOUTP_FDCTHCMAPTCWarningSta_flg_ovrdval
  VTHC_FDCompCmd_rpm_Inproc : FVT_lib/outp/OverrideAndLimit  SystemSampleTime=-1  VariantActivationTime=update diagram  Latency=0  AutoFrameSizeCalculation=off
      link override Signal_Limit/_maxval: Value=KOUTP_FDCompCmd_rpm_maxval
      link override Signal_Limit/_minval: Value=KOUTP_FDCompCmd_rpm_minval
      link override Signal_Override/_ovrdflg: Value=KOUTP_FDCompCmd_rpm_ovrdflg
      link override Signal_Override/_ovrdval: Value=KOUTP_FDCompCmd_rpm_ovrdval
  VTHC_FDEWP1Cmd_enum_Inproc : FVT_lib/outp/OverrideAndLimit  SystemSampleTime=-1  VariantActivationTime=update diagram  Latency=0  AutoFrameSizeCalculation=off
      link override Signal_Limit/_maxval: Value=KOUTP_FDEWP1Cmd_enum_maxval
      link override Signal_Limit/_minval: Value=KOUTP_FDEWP1Cmd_enum_minval
      link override Signal_Override/_ovrdflg: Value=KOUTP_FDEWP1Cmd_enum_ovrdflg
      link override Signal_Override/_ovrdval: Value=KOUTP_FDEWP1Cmd_enum_ovrdval
  VTHC_FDEWP2Cmd_enum_Inproc : FVT_lib/outp/OverrideAndLimit  SystemSampleTime=-1  VariantActivationTime=update diagram  Latency=0  AutoFrameSizeCalculation=off
      link override Signal_Limit/_maxval: Value=KOUTP_FDEWP2Cmd_enum_maxval
      link override Signal_Limit/_minval: Value=KOUTP_FDEWP2Cmd_enum_minval
      link override Signal_Override/_ovrdflg: Value=KOUTP_FDEWP2Cmd_enum_ovrdflg
      link override Signal_Override/_ovrdval: Value=KOUTP_FDEWP2Cmd_enum_ovrdval
  VTHC_FDEWP3Cmd_enum_Inproc : FVT_lib/outp/OverrideAndLimit  SystemSampleTime=-1  VariantActivationTime=update diagram  Latency=0  AutoFrameSizeCalculation=off
      link override Signal_Limit/_maxval: Value=KOUTP_FDEWP3Cmd_enum_maxval
      link override Signal_Limit/_minval: Value=KOUTP_FDEWP3Cmd_enum_minval
      link override Signal_Override/_ovrdflg: Value=KOUTP_FDEWP3Cmd_enum_ovrdflg
      link override Signal_Override/_ovrdval: Value=KOUTP_FDEWP3Cmd_enum_ovrdval
  VTHC_FDEXV1Cmd_step_Inproc : FVT_lib/outp/OverrideAndLimit  SystemSampleTime=-1  VariantActivationTime=update diagram  Latency=0  AutoFrameSizeCalculation=off
      link override Signal_Limit/_maxval: Value=KOUTP_FDEXV1Cmd_step_maxval
      link override Signal_Limit/_minval: Value=KOUTP_FDEXV1Cmd_step_minval
      link override Signal_Override/_ovrdflg: Value=KOUTP_FDEXV1Cmd_step_ovrdflg
      link override Signal_Override/_ovrdval: Value=KOUTP_FDEXV1Cmd_step_ovrdval
  VTHC_FDEXV2Cmd_step_Inproc : FVT_lib/outp/OverrideAndLimit  SystemSampleTime=-1  VariantActivationTime=update diagram  Latency=0  AutoFrameSizeCalculation=off
      link override Signal_Limit/_maxval: Value=KOUTP_FDEXV2Cmd_step_maxval
      link override Signal_Limit/_minval: Value=KOUTP_FDEXV2Cmd_step_minval
      link override Signal_Override/_ovrdflg: Value=KOUTP_FDEXV2Cmd_step_ovrdflg
      link override Signal_Override/_ovrdval: Value=KOUTP_FDEXV2Cmd_step_ovrdval
  VTHC_FDFWVCmd_flg_Inproc : FVT_lib/outp/OverrideAndLimit  SystemSampleTime=-1  VariantActivationTime=update diagram  Latency=0  AutoFrameSizeCalculation=off
      link override Signal_Limit/_maxval: Value=KOUTP_FDFWVCmd_flg_maxval
      link override Signal_Limit/_minval: Value=KOUTP_FDFWVCmd_flg_minval
      link override Signal_Override/_ovrdflg: Value=KOUTP_FDFWVCmd_flg_ovrdflg
      link override Signal_Override/_ovrdval: Value=KOUTP_FDFWVCmd_flg_ovrdval
  VTHC_FDFrLeAPTCHeatPwrCmd_W_Inproc : FVT_lib/outp/OverrideAndLimit  SystemSampleTime=-1  VariantActivationTime=update diagram  Latency=0  AutoFrameSizeCalculation=off
      link override Signal_Limit/_maxval: Value=KOUTP_FDFrLeAPTCHeatPwrCmd_W_maxval
      link override Signal_Limit/_minval: Value=KOUTP_FDFrLeAPTCHeatPwrCmd_W_minval
      link override Signal_Override/_ovrdflg: Value=KOUTP_FDFrLeAPTCHeatPwrCmd_W_ovrdflg
      link override Signal_Override/_ovrdval: Value=KOUTP_FDFrLeAPTCHeatPwrCmd_W_ovrdval
  VTHC_FDFrRiAPTCHeatPwrCmd_W_Inproc : FVT_lib/outp/OverrideAndLimit  SystemSampleTime=-1  VariantActivationTime=update diagram  Latency=0  AutoFrameSizeCalculation=off
      link override Signal_Limit/_maxval: Value=KOUTP_FDFrRiAPTCHeatPwrCmd_W_maxval
      link override Signal_Limit/_minval: Value=KOUTP_FDFrRiAPTCHeatPwrCmd_W_minval
      link override Signal_Override/_ovrdflg: Value=KOUTP_FDFrRiAPTCHeatPwrCmd_W_ovrdflg
      link override Signal_Override/_ovrdval: Value=KOUTP_FDFrRiAPTCHeatPwrCmd_W_ovrdval
  VTHC_FDFrWPTCHeatPwrCmd_W_Inproc : FVT_lib/outp/OverrideAndLimit  SystemSampleTime=-1  VariantActivationTime=update diagram  Latency=0  AutoFrameSizeCalculation=off
      link override Signal_Limit/_maxval: Value=KOUTP_FDFrWPTCHeatPwrCmd_W_maxval
      link override Signal_Limit/_minval: Value=KOUTP_FDFrWPTCHeatPwrCmd_W_minval
      link override Signal_Override/_ovrdflg: Value=KOUTP_FDFrWPTCHeatPwrCmd_W_ovrdflg
      link override Signal_Override/_ovrdval: Value=KOUTP_FDFrWPTCHeatPwrCmd_W_ovrdval
  VTHC_FDRecyAutoCmd_enum_Inproc : FVT_lib/outp/OverrideAndLimit  SystemSampleTime=-1  VariantActivationTime=update diagram  Latency=0  AutoFrameSizeCalculation=off
      link override Signal_Limit/_maxval: Value=KOUTP_FDRecyAutoCmd_enum_maxval
      link override Signal_Limit/_minval: Value=KOUTP_FDRecyAutoCmd_enum_minval
      link override Signal_Override/_ovrdflg: Value=KOUTP_FDRecyAutoCmd_enum_ovrdflg
      link override Signal_Override/_ovrdval: Value=KOUTP_FDRecyAutoCmd_enum_ovrdval
  VTHC_FDRrAPTCHeatPwrCmd_W_Inproc : FVT_lib/outp/OverrideAndLimit  SystemSampleTime=-1  VariantActivationTime=update diagram  Latency=0  AutoFrameSizeCalculation=off
      link override Signal_Limit/_maxval: Value=KOUTP_FDRrAPTCHeatPwrCmd_W_maxval
      link override Signal_Limit/_minval: Value=KOUTP_FDRrAPTCHeatPwrCmd_W_minval
      link override Signal_Override/_ovrdflg: Value=KOUTP_FDRrAPTCHeatPwrCmd_W_ovrdflg
      link override Signal_Override/_ovrdval: Value=KOUTP_FDRrAPTCHeatPwrCmd_W_ovrdval
  VTHC_FDSOTXVCmd_flg_Inproc : FVT_lib/outp/OverrideAndLimit  SystemSampleTime=-1  VariantActivationTime=update diagram  Latency=0  AutoFrameSizeCalculation=off
      link override Signal_Limit/_maxval: Value=KOUTP_FDSOTXVCmd_flg_maxval
      link override Signal_Limit/_minval: Value=KOUTP_FDSOTXVCmd_flg_minval
      link override Signal_Override/_ovrdflg: Value=KOUTP_FDSOTXVCmd_flg_ovrdflg
      link override Signal_Override/_ovrdval: Value=KOUTP_FDSOTXVCmd_flg_ovrdval
  VTHC_FDSOV1Cmd_flg_Inproc : FVT_lib/outp/OverrideAndLimit  SystemSampleTime=-1  VariantActivationTime=update diagram  Latency=0  AutoFrameSizeCalculation=off
      link override Signal_Limit/_maxval: Value=KOUTP_FDSOV1Cmd_flg_maxval
      link override Signal_Limit/_minval: Value=KOUTP_FDSOV1Cmd_flg_minval
      link override Signal_Override/_ovrdflg: Value=KOUTP_FDSOV1Cmd_flg_ovrdflg
      link override Signal_Override/_ovrdval: Value=KOUTP_FDSOV1Cmd_flg_ovrdval
  VTHC_FDSOV2Cmd_flg_Inproc : FVT_lib/outp/OverrideAndLimit  SystemSampleTime=-1  VariantActivationTime=update diagram  Latency=0  AutoFrameSizeCalculation=off
      link override Signal_Limit/_maxval: Value=KOUTP_FDSOV2Cmd_flg_maxval
      link override Signal_Limit/_minval: Value=KOUTP_FDSOV2Cmd_flg_minval
      link override Signal_Override/_ovrdflg: Value=KOUTP_FDSOV2Cmd_flg_ovrdflg
      link override Signal_Override/_ovrdval: Value=KOUTP_FDSOV2Cmd_flg_ovrdval
  VTHC_FDSOV3Cmd_flg_Inproc : FVT_lib/outp/OverrideAndLimit  SystemSampleTime=-1  VariantActivationTime=update diagram  Latency=0  AutoFrameSizeCalculation=off
      link override Signal_Limit/_maxval: Value=KOUTP_FDSOV3Cmd_flg_maxval
      link override Signal_Limit/_minval: Value=KOUTP_FDSOV3Cmd_flg_minval
      link override Signal_Override/_ovrdflg: Value=KOUTP_FDSOV3Cmd_flg_ovrdflg
      link override Signal_Override/_ovrdval: Value=KOUTP_FDSOV3Cmd_flg_ovrdval
  VTHC_FDTWVCmd_pct_Inproc : FVT_lib/outp/OverrideAndLimit  SystemSampleTime=-1  VariantActivationTime=update diagram  Latency=0  AutoFrameSizeCalculation=off
      link override Signal_Limit/_maxval: Value=KOUTP_FDTWVCmd_pct_maxval
      link override Signal_Limit/_minval: Value=KOUTP_FDTWVCmd_pct_minval
      link override Signal_Override/_ovrdflg: Value=KOUTP_FDTWVCmd_pct_ovrdflg
      link override Signal_Override/_ovrdval: Value=KOUTP_FDTWVCmd_pct_ovrdval
  VTHC_FaceM_flg_Inproc : FVT_lib/outp/OverrideAndLimit  SystemSampleTime=-1  VariantActivationTime=update diagram  Latency=0  AutoFrameSizeCalculation=off
      link override Signal_Limit/_maxval: Value=KOUTP_FaceM_flg_maxval
      link override Signal_Limit/_minval: Value=KOUTP_FaceM_flg_minval
      link override Signal_Override/_ovrdflg: Value=KOUTP_FaceM_flg_ovrdflg
      link override Signal_Override/_ovrdval: Value=KOUTP_FaceM_flg_ovrdval
  VTHC_Face_flg_Inproc : FVT_lib/outp/OverrideAndLimit  SystemSampleTime=-1  VariantActivationTime=update diagram  Latency=0  AutoFrameSizeCalculation=off
      link override Signal_Limit/_maxval: Value=KOUTP_Face_flg_maxval
      link override Signal_Limit/_minval: Value=KOUTP_Face_flg_minval
      link override Signal_Override/_ovrdflg: Value=KOUTP_Face_flg_ovrdflg
      link override Signal_Override/_ovrdval: Value=KOUTP_Face_flg_ovrdval
  VTHC_FootM_flg_Inproc : FVT_lib/outp/OverrideAndLimit  SystemSampleTime=-1  VariantActivationTime=update diagram  Latency=0  AutoFrameSizeCalculation=off
      link override Signal_Limit/_maxval: Value=KOUTP_FootM_flg_maxval
      link override Signal_Limit/_minval: Value=KOUTP_FootM_flg_minval
      link override Signal_Override/_ovrdflg: Value=KOUTP_FootM_flg_ovrdflg
      link override Signal_Override/_ovrdval: Value=KOUTP_FootM_flg_ovrdval
  VTHC_Foot_flg_Inproc : FVT_lib/outp/OverrideAndLimit  SystemSampleTime=-1  VariantActivationTime=update diagram  Latency=0  AutoFrameSizeCalculation=off
      link override Signal_Limit/_maxval: Value=KOUTP_Foot_flg_maxval
      link override Signal_Limit/_minval: Value=KOUTP_Foot_flg_minval
      link override Signal_Override/_ovrdflg: Value=KOUTP_Foot_flg_ovrdflg
      link override Signal_Override/_ovrdval: Value=KOUTP_Foot_flg_ovrdval
  VTHC_Frost_flg_Inproc : FVT_lib/outp/OverrideAndLimit  SystemSampleTime=-1  VariantActivationTime=update diagram  Latency=0  AutoFrameSizeCalculation=off
      link override Signal_Limit/_maxval: Value=KOUTP_Frost_flg_maxval
      link override Signal_Limit/_minval: Value=KOUTP_Frost_flg_minval
      link override Signal_Override/_ovrdflg: Value=KOUTP_Frost_flg_ovrdflg
      link override Signal_Override/_ovrdval: Value=KOUTP_Frost_flg_ovrdval
  VTHC_RecAutoFlg_flg_Inproc : FVT_lib/outp/OverrideAndLimit  SystemSampleTime=-1  VariantActivationTime=update diagram  Latency=0  AutoFrameSizeCalculation=off
      link override Signal_Limit/_maxval: Value=KOUTP_RecAutoFlg_flg_maxval
      link override Signal_Limit/_minval: Value=KOUTP_RecAutoFlg_flg_minval
      link override Signal_Override/_ovrdflg: Value=KOUTP_RecAutoFlg_flg_ovrdflg
      link override Signal_Override/_ovrdval: Value=KOUTP_RecAutoFlg_flg_ovrdval
  VTHC_fdefog_flg_Inproc : FVT_lib/outp/OverrideAndLimit  SystemSampleTime=-1  VariantActivationTime=update diagram  Latency=0  AutoFrameSizeCalculation=off
      link override Signal_Limit/_maxval: Value=KOUTP_fdefog_flg_maxval
      link override Signal_Limit/_minval: Value=KOUTP_fdefog_flg_minval
      link override Signal_Override/_ovrdflg: Value=KOUTP_fdefog_flg_ovrdflg
      link override Signal_Override/_ovrdval: Value=KOUTP_fdefog_flg_ovrdval
  VTHC_sigAirIntenZon1St_enum_Inproc : FVT_lib/outp/OverrideAndLimit  SystemSampleTime=-1  VariantActivationTime=update diagram  Latency=0  AutoFrameSizeCalculation=off
      link override Signal_Limit/_maxval: Value=KOUTP_sigAirIntenZon1St_enum_maxval
      link override Signal_Limit/_minval: Value=KOUTP_sigAirIntenZon1St_enum_minval
      link override Signal_Override/_ovrdflg: Value=KOUTP_sigAirIntenZon1St_enum_ovrdflg
      link override Signal_Override/_ovrdval: Value=KOUTP_sigAirIntenZon1St_enum_ovrdval
  VTHC_sigAmbAirT_C_Inproc : FVT_lib/outp/OverrideAndLimit  SystemSampleTime=-1  VariantActivationTime=update diagram  Latency=0  AutoFrameSizeCalculation=off
      link override Signal_Limit/_maxval: Value=KOUTP_sigAmbAirT_C_maxval
      link override Signal_Limit/_minval: Value=KOUTP_sigAmbAirT_C_minval
      link override Signal_Override/_ovrdflg: Value=KOUTP_sigAmbAirT_C_ovrdflg
      link override Signal_Override/_ovrdval: Value=KOUTP_sigAmbAirT_C_ovrdval
  VTHC_sigCbnAirT_C_Inproc : FVT_lib/outp/OverrideAndLimit  SystemSampleTime=-1  VariantActivationTime=update diagram  Latency=0  AutoFrameSizeCalculation=off
      link override Signal_Limit/_maxval: Value=KOUTP_sigCbnAirT_C_maxval
      link override Signal_Limit/_minval: Value=KOUTP_sigCbnAirT_C_minval
      link override Signal_Override/_ovrdflg: Value=KOUTP_sigCbnAirT_C_ovrdflg
      link override Signal_Override/_ovrdval: Value=KOUTP_sigCbnAirT_C_ovrdval
  VTHC_sigCbnSolarLeft_W_Inproc : FVT_lib/outp/OverrideAndLimit  SystemSampleTime=-1  VariantActivationTime=update diagram  Latency=0  AutoFrameSizeCalculation=off
      link override Signal_Limit/_maxval: Value=KOUTP_sigCbnSolarLeft_W_maxval
      link override Signal_Limit/_minval: Value=KOUTP_sigCbnSolarLeft_W_minval
      link override Signal_Override/_ovrdflg: Value=KOUTP_sigCbnSolarLeft_W_ovrdflg
      link override Signal_Override/_ovrdval: Value=KOUTP_sigCbnSolarLeft_W_ovrdval
  VTHC_sigCbnSolarRight_W_Inproc : FVT_lib/outp/OverrideAndLimit  SystemSampleTime=-1  VariantActivationTime=update diagram  Latency=0  AutoFrameSizeCalculation=off
      link override Signal_Limit/_maxval: Value=KOUTP_sigCbnSolarRight_W_maxval
      link override Signal_Limit/_minval: Value=KOUTP_sigCbnSolarRight_W_minval
      link override Signal_Override/_ovrdflg: Value=KOUTP_sigCbnSolarRight_W_ovrdflg
      link override Signal_Override/_ovrdval: Value=KOUTP_sigCbnSolarRight_W_ovrdval
  VTHC_sigClntTHvBattIn_C_Inproc : FVT_lib/outp/OverrideAndLimit  SystemSampleTime=-1  VariantActivationTime=update diagram  Latency=0  AutoFrameSizeCalculation=off
      link override Signal_Limit/_maxval: Value=KOUTP_sigClntTHvBattIn_C_maxval
      link override Signal_Limit/_minval: Value=KOUTP_sigClntTHvBattIn_C_minval
      link override Signal_Override/_ovrdflg: Value=KOUTP_sigClntTHvBattIn_C_ovrdflg
      link override Signal_Override/_ovrdval: Value=KOUTP_sigClntTHvBattIn_C_ovrdval
  VTHC_sigClntTHvBattOut_C_Inproc : FVT_lib/outp/OverrideAndLimit  SystemSampleTime=-1  VariantActivationTime=update diagram  Latency=0  AutoFrameSizeCalculation=off
      link override Signal_Limit/_maxval: Value=KOUTP_sigClntTHvBattOut_C_maxval
      link override Signal_Limit/_minval: Value=KOUTP_sigClntTHvBattOut_C_minval
      link override Signal_Override/_ovrdflg: Value=KOUTP_sigClntTHvBattOut_C_ovrdflg
      link override Signal_Override/_ovrdval: Value=KOUTP_sigClntTHvBattOut_C_ovrdval
  VTHC_sigRecircSt_flg_Inproc : FVT_lib/outp/OverrideAndLimit  SystemSampleTime=-1  VariantActivationTime=update diagram  Latency=0  AutoFrameSizeCalculation=off
      link override Signal_Limit/_maxval: Value=KOUTP_sigRecircSt_flg_maxval
      link override Signal_Limit/_minval: Value=KOUTP_sigRecircSt_flg_minval
      link override Signal_Override/_ovrdflg: Value=KOUTP_sigRecircSt_flg_ovrdflg
      link override Signal_Override/_ovrdval: Value=KOUTP_sigRecircSt_flg_ovrdval
  VTHC_sigSetTempZon1St_C_Inproc : FVT_lib/outp/OverrideAndLimit  SystemSampleTime=-1  VariantActivationTime=update diagram  Latency=0  AutoFrameSizeCalculation=off
      link override Signal_Limit/_maxval: Value=KOUTP_sigSetTempZon1St_C_maxval
      link override Signal_Limit/_minval: Value=KOUTP_sigSetTempZon1St_C_minval
      link override Signal_Override/_ovrdflg: Value=KOUTP_sigSetTempZon1St_C_ovrdflg
      link override Signal_Override/_ovrdval: Value=KOUTP_sigSetTempZon1St_C_ovrdval
  VTHC_sigSetTempZon2StM_C_Inproc : FVT_lib/outp/OverrideAndLimit  SystemSampleTime=-1  VariantActivationTime=update diagram  Latency=0  AutoFrameSizeCalculation=off
      link override Signal_Limit/_maxval: Value=KOUTP_sigSetTempZon2StM_C_maxval
      link override Signal_Limit/_minval: Value=KOUTP_sigSetTempZon2StM_C_minval
      link override Signal_Override/_ovrdflg: Value=KOUTP_sigSetTempZon2StM_C_ovrdflg
      link override Signal_Override/_ovrdval: Value=KOUTP_sigSetTempZon2StM_C_ovrdval
  VTHC_sigSetTempZon2St_C_Inproc : FVT_lib/outp/OverrideAndLimit  SystemSampleTime=-1  VariantActivationTime=update diagram  Latency=0  AutoFrameSizeCalculation=off
      link override Signal_Limit/_maxval: Value=KOUTP_sigSetTempZon2St_C_maxval
      link override Signal_Limit/_minval: Value=KOUTP_sigSetTempZon2St_C_minval
      link override Signal_Override/_ovrdflg: Value=KOUTP_sigSetTempZon2St_C_ovrdflg
      link override Signal_Override/_ovrdval: Value=KOUTP_sigSetTempZon2St_C_ovrdval
  VTHC_sigWindDirZon1St_enum_Inproc : FVT_lib/outp/OverrideAndLimit  SystemSampleTime=-1  VariantActivationTime=update diagram  Latency=0  AutoFrameSizeCalculation=off
      link override Signal_Limit/_maxval: Value=KOUTP_sigWindDirZon1St_enum_maxval
      link override Signal_Limit/_minval: Value=KOUTP_sigWindDirZon1St_enum_minval
      link override Signal_Override/_ovrdflg: Value=KOUTP_sigWindDirZon1St_enum_ovrdflg
      link override Signal_Override/_ovrdval: Value=KOUTP_sigWindDirZon1St_enum_ovrdval
  VTPM_ALFin_flg_Inproc : FVT_lib/outp/OverrideAndLimit  SystemSampleTime=-1  VariantActivationTime=update diagram  Latency=0  AutoFrameSizeCalculation=off
      link override Signal_Limit/_maxval: Value=KOUTP_ALFin_flg_maxval
      link override Signal_Limit/_minval: Value=KOUTP_ALFin_flg_minval
      link override Signal_Override/_ovrdflg: Value=KOUTP_ALFin_flg_ovrdflg
      link override Signal_Override/_ovrdval: Value=KOUTP_ALFin_flg_ovrdval
  VTPM_AutoLTips_enum_Inproc : FVT_lib/outp/OverrideAndLimit  SystemSampleTime=-1  VariantActivationTime=update diagram  Latency=0  AutoFrameSizeCalculation=off
      link override Signal_Limit/_maxval: Value=KOUTP_AutoLTips_enum_maxval
      link override Signal_Limit/_minval: Value=KOUTP_AutoLTips_enum_minval
      link override Signal_Override/_ovrdflg: Value=KOUTP_AutoLTips_enum_ovrdflg
      link override Signal_Override/_ovrdval: Value=KOUTP_AutoLTips_enum_ovrdval
  VTPM_CWheelTips_enum_Inproc : FVT_lib/outp/OverrideAndLimit  SystemSampleTime=-1  VariantActivationTime=update diagram  Latency=0  AutoFrameSizeCalculation=off
      link override Signal_Limit/_maxval: Value=KOUTP_CWheelTips_enum_maxval
      link override Signal_Limit/_minval: Value=KOUTP_CWheelTips_enum_minval
      link override Signal_Override/_ovrdflg: Value=KOUTP_CWheelTips_enum_ovrdflg
      link override Signal_Override/_ovrdval: Value=KOUTP_CWheelTips_enum_ovrdval
  VTPM_ChkStorge_flg_Inproc : FVT_lib/outp/OverrideAndLimit  SystemSampleTime=-1  VariantActivationTime=update diagram  Latency=0  AutoFrameSizeCalculation=off
      link override Signal_Limit/_maxval: Value=KOUTP_ChkStorge_flg_maxval
      link override Signal_Limit/_minval: Value=KOUTP_ChkStorge_flg_minval
      link override Signal_Override/_ovrdflg: Value=KOUTP_ChkStorge_flg_ovrdflg
      link override Signal_Override/_ovrdval: Value=KOUTP_ChkStorge_flg_ovrdval
  VTPM_Chkfin_flg_Inproc : FVT_lib/outp/OverrideAndLimit  SystemSampleTime=-1  VariantActivationTime=update diagram  Latency=0  AutoFrameSizeCalculation=off
      link override Signal_Limit/_maxval: Value=KOUTP_Chkfin_flg_maxval
      link override Signal_Limit/_minval: Value=KOUTP_Chkfin_flg_minval
      link override Signal_Override/_ovrdflg: Value=KOUTP_Chkfin_flg_ovrdflg
      link override Signal_Override/_ovrdval: Value=KOUTP_Chkfin_flg_ovrdval
  VTPM_FAT_flg_Inproc : FVT_lib/outp/OverrideAndLimit  SystemSampleTime=-1  VariantActivationTime=update diagram  Latency=0  AutoFrameSizeCalculation=off
      link override Signal_Limit/_maxval: Value=KOUTP_FAT_flg_maxval
      link override Signal_Limit/_minval: Value=KOUTP_FAT_flg_minval
      link override Signal_Override/_ovrdflg: Value=KOUTP_FAT_flg_ovrdflg
      link override Signal_Override/_ovrdval: Value=KOUTP_FAT_flg_ovrdval
  VTPM_FlashIDvalid_enum_Inproc : FVT_lib/outp/OverrideAndLimit  SystemSampleTime=-1  VariantActivationTime=update diagram  Latency=0  AutoFrameSizeCalculation=off
      link override Signal_Limit/_maxval: Value=KOUTP_FlashIDvalid_enum_maxval
      link override Signal_Limit/_minval: Value=KOUTP_FlashIDvalid_enum_minval
      link override Signal_Override/_ovrdflg: Value=KOUTP_FlashIDvalid_enum_ovrdflg
      link override Signal_Override/_ovrdval: Value=KOUTP_FlashIDvalid_enum_ovrdval
  VTPM_FlashS1ID_raw_Inproc : FVT_lib/outp/OverrideAndLimit  SystemSampleTime=-1  VariantActivationTime=update diagram  Latency=0  AutoFrameSizeCalculation=off
      link override Signal_Limit/_maxval: Value=KOUTP_FlashS1ID_raw_maxval
      link override Signal_Limit/_minval: Value=KOUTP_FlashS1ID_raw_minval
      link override Signal_Override/_ovrdflg: Value=KOUTP_FlashS1ID_raw_ovrdflg
      link override Signal_Override/_ovrdval: Value=KOUTP_FlashS1ID_raw_ovrdval
  VTPM_FlashS2ID_raw_Inproc : FVT_lib/outp/OverrideAndLimit  SystemSampleTime=-1  VariantActivationTime=update diagram  Latency=0  AutoFrameSizeCalculation=off
      link override Signal_Limit/_maxval: Value=KOUTP_FlashS2ID_raw_maxval
      link override Signal_Limit/_minval: Value=KOUTP_FlashS2ID_raw_minval
      link override Signal_Override/_ovrdflg: Value=KOUTP_FlashS2ID_raw_ovrdflg
      link override Signal_Override/_ovrdval: Value=KOUTP_FlashS2ID_raw_ovrdval
  VTPM_FlashS3ID_raw_Inproc : FVT_lib/outp/OverrideAndLimit  SystemSampleTime=-1  VariantActivationTime=update diagram  Latency=0  AutoFrameSizeCalculation=off
      link override Signal_Limit/_maxval: Value=KOUTP_FlashS3ID_raw_maxval
      link override Signal_Limit/_minval: Value=KOUTP_FlashS3ID_raw_minval
      link override Signal_Override/_ovrdflg: Value=KOUTP_FlashS3ID_raw_ovrdflg
      link override Signal_Override/_ovrdval: Value=KOUTP_FlashS3ID_raw_ovrdval
  VTPM_FlashS4ID_raw_Inproc : FVT_lib/outp/OverrideAndLimit  SystemSampleTime=-1  VariantActivationTime=update diagram  Latency=0  AutoFrameSizeCalculation=off
      link override Signal_Limit/_maxval: Value=KOUTP_FlashS4ID_raw_maxval
      link override Signal_Limit/_minval: Value=KOUTP_FlashS4ID_raw_minval
      link override Signal_Override/_ovrdflg: Value=KOUTP_FlashS4ID_raw_ovrdflg
      link override Signal_Override/_ovrdval: Value=KOUTP_FlashS4ID_raw_ovrdval
  VTPM_Flashchkdatavalid_enum_Inproc : FVT_lib/outp/OverrideAndLimit  SystemSampleTime=-1  VariantActivationTime=update diagram  Latency=0  AutoFrameSizeCalculation=off
      link override Signal_Limit/_maxval: Value=KOUTP_Flashchkdatavalid_enum_maxval
      link override Signal_Limit/_minval: Value=KOUTP_Flashchkdatavalid_enum_minval
      link override Signal_Override/_ovrdflg: Value=KOUTP_Flashchkdatavalid_enum_ovrdflg
      link override Signal_Override/_ovrdval: Value=KOUTP_Flashchkdatavalid_enum_ovrdval
  VTPM_Flashdatavalid_enum_Inproc : FVT_lib/outp/OverrideAndLimit  SystemSampleTime=-1  VariantActivationTime=update diagram  Latency=0  AutoFrameSizeCalculation=off
      link override Signal_Limit/_maxval: Value=KOUTP_Flashdatavalid_enum_maxval
      link override Signal_Limit/_minval: Value=KOUTP_Flashdatavalid_enum_minval
      link override Signal_Override/_ovrdflg: Value=KOUTP_Flashdatavalid_enum_ovrdflg
      link override Signal_Override/_ovrdval: Value=KOUTP_Flashdatavalid_enum_ovrdval
  VTPM_ID1messageALTU_raw8_Inproc : FVT_lib/outp/OverrideAndLimit  SystemSampleTime=-1  VariantActivationTime=update diagram  Latency=0  AutoFrameSizeCalculation=off
      link override Signal_Limit/_maxval: Value=KOUTP_ID1messageALTU_raw8_maxval
      link override Signal_Limit/_minval: Value=KOUTP_ID1messageALTU_raw8_minval
      link override Signal_Override/_ovrdflg: Value=KOUTP_ID1messageALTU_raw8_ovrdflg
      link override Signal_Override/_ovrdval: Value=KOUTP_ID1messageALTU_raw8_ovrdval
  VTPM_ID2messageALTU_raw8_Inproc : FVT_lib/outp/OverrideAndLimit  SystemSampleTime=-1  VariantActivationTime=update diagram  Latency=0  AutoFrameSizeCalculation=off
      link override Signal_Limit/_maxval: Value=KOUTP_ID2messageALTU_raw8_maxval
      link override Signal_Limit/_minval: Value=KOUTP_ID2messageALTU_raw8_minval
      link override Signal_Override/_ovrdflg: Value=KOUTP_ID2messageALTU_raw8_ovrdflg
      link override Signal_Override/_ovrdval: Value=KOUTP_ID2messageALTU_raw8_ovrdval
  VTPM_ID3messageALTU_raw8_Inproc : FVT_lib/outp/OverrideAndLimit  SystemSampleTime=-1  VariantActivationTime=update diagram  Latency=0  AutoFrameSizeCalculation=off
      link override Signal_Limit/_maxval: Value=KOUTP_ID3messageALTU_raw8_maxval
      link override Signal_Limit/_minval: Value=KOUTP_ID3messageALTU_raw8_minval
      link override Signal_Override/_ovrdflg: Value=KOUTP_ID3messageALTU_raw8_ovrdflg
      link override Signal_Override/_ovrdval: Value=KOUTP_ID3messageALTU_raw8_ovrdval
  VTPM_ID4messageALTU_raw8_Inproc : FVT_lib/outp/OverrideAndLimit  SystemSampleTime=-1  VariantActivationTime=update diagram  Latency=0  AutoFrameSizeCalculation=off
      link override Signal_Limit/_maxval: Value=KOUTP_ID4messageALTU_raw8_maxval
      link override Signal_Limit/_minval: Value=KOUTP_ID4messageALTU_raw8_minval
      link override Signal_Override/_ovrdflg: Value=KOUTP_ID4messageALTU_raw8_ovrdflg
      link override Signal_Override/_ovrdval: Value=KOUTP_ID4messageALTU_raw8_ovrdval
  VTPM_IDin_raw32_Inproc : FVT_lib/outp/OverrideAndLimit  SystemSampleTime=-1  VariantActivationTime=update diagram  Latency=0  AutoFrameSizeCalculation=off
      link override Signal_Limit/_maxval: Value=KOUTP_IDin_raw32_maxval
      link override Signal_Limit/_minval: Value=KOUTP_IDin_raw32_minval
      link override Signal_Override/_ovrdflg: Value=KOUTP_IDin_raw32_ovrdflg
      link override Signal_Override/_ovrdval: Value=KOUTP_IDin_raw32_ovrdval
  VTPM_LFBatWarn_flg_Inproc : FVT_lib/outp/OverrideAndLimit  SystemSampleTime=-1  VariantActivationTime=update diagram  Latency=0  AutoFrameSizeCalculation=off
      link override Signal_Limit/_maxval: Value=KOUTP_LFBatWarn_flg_maxval
      link override Signal_Limit/_minval: Value=KOUTP_LFBatWarn_flg_minval
      link override Signal_Override/_ovrdflg: Value=KOUTP_LFBatWarn_flg_ovrdflg
      link override Signal_Override/_ovrdval: Value=KOUTP_LFBatWarn_flg_ovrdval
  VTPM_LFP20_raw8_Inproc : FVT_lib/outp/OverrideAndLimit  SystemSampleTime=-1  VariantActivationTime=update diagram  Latency=0  AutoFrameSizeCalculation=off
      link override Signal_Limit/_maxval: Value=KOUTP_LFP20_raw8_maxval
      link override Signal_Limit/_minval: Value=KOUTP_LFP20_raw8_minval
      link override Signal_Override/_ovrdflg: Value=KOUTP_LFP20_raw8_ovrdflg
      link override Signal_Override/_ovrdval: Value=KOUTP_LFP20_raw8_ovrdval
  VTPM_LFPindi_enum_Inproc : FVT_lib/outp/OverrideAndLimit  SystemSampleTime=-1  VariantActivationTime=update diagram  Latency=0  AutoFrameSizeCalculation=off
      link override Signal_Limit/_maxval: Value=KOUTP_LFPindi_enum_maxval
      link override Signal_Limit/_minval: Value=KOUTP_LFPindi_enum_minval
      link override Signal_Override/_ovrdflg: Value=KOUTP_LFPindi_enum_ovrdflg
      link override Signal_Override/_ovrdval: Value=KOUTP_LFPindi_enum_ovrdval
  VTPM_LFPressIndi_enum_Inproc : FVT_lib/outp/OverrideAndLimit  SystemSampleTime=-1  VariantActivationTime=update diagram  Latency=0  AutoFrameSizeCalculation=off
      link override Signal_Limit/_maxval: Value=KOUTP_LFPressIndi_enum_maxval
      link override Signal_Limit/_minval: Value=KOUTP_LFPressIndi_enum_minval
      link override Signal_Override/_ovrdflg: Value=KOUTP_LFPressIndi_enum_ovrdflg
      link override Signal_Override/_ovrdval: Value=KOUTP_LFPressIndi_enum_ovrdval
  VTPM_LFSensorFail_flg_Inproc : FVT_lib/outp/OverrideAndLimit  SystemSampleTime=-1  VariantActivationTime=update diagram  Latency=0  AutoFrameSizeCalculation=off
      link override Signal_Limit/_maxval: Value=KOUTP_LFSensorFail_flg_maxval
      link override Signal_Limit/_minval: Value=KOUTP_LFSensorFail_flg_minval
      link override Signal_Override/_ovrdflg: Value=KOUTP_LFSensorFail_flg_ovrdflg
      link override Signal_Override/_ovrdval: Value=KOUTP_LFSensorFail_flg_ovrdval
  VTPM_LFSensorMode_flg_Inproc : FVT_lib/outp/OverrideAndLimit  SystemSampleTime=-1  VariantActivationTime=update diagram  Latency=0  AutoFrameSizeCalculation=off
      link override Signal_Limit/_maxval: Value=KOUTP_LFSensorMode_flg_maxval
      link override Signal_Limit/_minval: Value=KOUTP_LFSensorMode_flg_minval
      link override Signal_Override/_ovrdflg: Value=KOUTP_LFSensorMode_flg_ovrdflg
      link override Signal_Override/_ovrdval: Value=KOUTP_LFSensorMode_flg_ovrdval
  VTPM_LFWheelDebug_flg_Inproc : FVT_lib/outp/OverrideAndLimit  SystemSampleTime=-1  VariantActivationTime=update diagram  Latency=0  AutoFrameSizeCalculation=off
      link override Signal_Limit/_maxval: Value=KOUTP_LFWheelDebug_flg_maxval
      link override Signal_Limit/_minval: Value=KOUTP_LFWheelDebug_flg_minval
      link override Signal_Override/_ovrdflg: Value=KOUTP_LFWheelDebug_flg_ovrdflg
      link override Signal_Override/_ovrdval: Value=KOUTP_LFWheelDebug_flg_ovrdval
  VTPM_LFWheelPSW_raw8_Inproc : FVT_lib/outp/OverrideAndLimit  SystemSampleTime=-1  VariantActivationTime=update diagram  Latency=0  AutoFrameSizeCalculation=off
      link override Signal_Limit/_maxval: Value=KOUTP_LFWheelPSW_raw8_maxval
      link override Signal_Limit/_minval: Value=KOUTP_LFWheelPSW_raw8_minval
      link override Signal_Override/_ovrdflg: Value=KOUTP_LFWheelPSW_raw8_ovrdflg
      link override Signal_Override/_ovrdval: Value=KOUTP_LFWheelPSW_raw8_ovrdval
  VTPM_LFWheelPress_raw8_Inproc : FVT_lib/outp/OverrideAndLimit  SystemSampleTime=-1  VariantActivationTime=update diagram  Latency=0  AutoFrameSizeCalculation=off
      link override Signal_Limit/_maxval: Value=KOUTP_LFWheelPress_raw8_maxval
      link override Signal_Limit/_minval: Value=KOUTP_LFWheelPress_raw8_minval
      link override Signal_Override/_ovrdflg: Value=KOUTP_LFWheelPress_raw8_ovrdflg
      link override Signal_Override/_ovrdval: Value=KOUTP_LFWheelPress_raw8_ovrdval
  VTPM_LFWheelTemp_C_Inproc : FVT_lib/outp/OverrideAndLimit  SystemSampleTime=-1  VariantActivationTime=update diagram  Latency=0  AutoFrameSizeCalculation=off
      link override Signal_Limit/_maxval: Value=KOUTP_LFWheelTemp_C_maxval
      link override Signal_Limit/_minval: Value=KOUTP_LFWheelTemp_C_minval
      link override Signal_Override/_ovrdflg: Value=KOUTP_LFWheelTemp_C_ovrdflg
      link override Signal_Override/_ovrdval: Value=KOUTP_LFWheelTemp_C_ovrdval
  VTPM_LFWheelTmpIndi_flg_Inproc : FVT_lib/outp/OverrideAndLimit  SystemSampleTime=-1  VariantActivationTime=update diagram  Latency=0  AutoFrameSizeCalculation=off
      link override Signal_Limit/_maxval: Value=KOUTP_LFWheelTmpIndi_flg_maxval
      link override Signal_Limit/_minval: Value=KOUTP_LFWheelTmpIndi_flg_minval
      link override Signal_Override/_ovrdflg: Value=KOUTP_LFWheelTmpIndi_flg_ovrdflg
      link override Signal_Override/_ovrdval: Value=KOUTP_LFWheelTmpIndi_flg_ovrdval
  VTPM_LRBatWarn_flg_Inproc : FVT_lib/outp/OverrideAndLimit  SystemSampleTime=-1  VariantActivationTime=update diagram  Latency=0  AutoFrameSizeCalculation=off
      link override Signal_Limit/_maxval: Value=KOUTP_LRBatWarn_flg_maxval
      link override Signal_Limit/_minval: Value=KOUTP_LRBatWarn_flg_minval
      link override Signal_Override/_ovrdflg: Value=KOUTP_LRBatWarn_flg_ovrdflg
      link override Signal_Override/_ovrdval: Value=KOUTP_LRBatWarn_flg_ovrdval
  VTPM_LRP20_raw8_Inproc : FVT_lib/outp/OverrideAndLimit  SystemSampleTime=-1  VariantActivationTime=update diagram  Latency=0  AutoFrameSizeCalculation=off
      link override Signal_Limit/_maxval: Value=KOUTP_LRP20_raw8_maxval
      link override Signal_Limit/_minval: Value=KOUTP_LRP20_raw8_minval
      link override Signal_Override/_ovrdflg: Value=KOUTP_LRP20_raw8_ovrdflg
      link override Signal_Override/_ovrdval: Value=KOUTP_LRP20_raw8_ovrdval
  VTPM_LRPindi_enum_Inproc : FVT_lib/outp/OverrideAndLimit  SystemSampleTime=-1  VariantActivationTime=update diagram  Latency=0  AutoFrameSizeCalculation=off
      link override Signal_Limit/_maxval: Value=KOUTP_LRPindi_enum_maxval
      link override Signal_Limit/_minval: Value=KOUTP_LRPindi_enum_minval
      link override Signal_Override/_ovrdflg: Value=KOUTP_LRPindi_enum_ovrdflg
      link override Signal_Override/_ovrdval: Value=KOUTP_LRPindi_enum_ovrdval
  VTPM_LRPressIndi_enum_Inproc : FVT_lib/outp/OverrideAndLimit  SystemSampleTime=-1  VariantActivationTime=update diagram  Latency=0  AutoFrameSizeCalculation=off
      link override Signal_Limit/_maxval: Value=KOUTP_LRPressIndi_enum_maxval
      link override Signal_Limit/_minval: Value=KOUTP_LRPressIndi_enum_minval
      link override Signal_Override/_ovrdflg: Value=KOUTP_LRPressIndi_enum_ovrdflg
      link override Signal_Override/_ovrdval: Value=KOUTP_LRPressIndi_enum_ovrdval
  VTPM_LRSensorFail_flg_Inproc : FVT_lib/outp/OverrideAndLimit  SystemSampleTime=-1  VariantActivationTime=update diagram  Latency=0  AutoFrameSizeCalculation=off
      link override Signal_Limit/_maxval: Value=KOUTP_LRSensorFail_flg_maxval
      link override Signal_Limit/_minval: Value=KOUTP_LRSensorFail_flg_minval
      link override Signal_Override/_ovrdflg: Value=KOUTP_LRSensorFail_flg_ovrdflg
      link override Signal_Override/_ovrdval: Value=KOUTP_LRSensorFail_flg_ovrdval
  VTPM_LRSensorMode_flg_Inproc : FVT_lib/outp/OverrideAndLimit  SystemSampleTime=-1  VariantActivationTime=update diagram  Latency=0  AutoFrameSizeCalculation=off
      link override Signal_Limit/_maxval: Value=KOUTP_LRSensorMode_flg_maxval
      link override Signal_Limit/_minval: Value=KOUTP_LRSensorMode_flg_minval
      link override Signal_Override/_ovrdflg: Value=KOUTP_LRSensorMode_flg_ovrdflg
      link override Signal_Override/_ovrdval: Value=KOUTP_LRSensorMode_flg_ovrdval
  VTPM_LRWheelDebug_flg_Inproc : FVT_lib/outp/OverrideAndLimit  SystemSampleTime=-1  VariantActivationTime=update diagram  Latency=0  AutoFrameSizeCalculation=off
      link override Signal_Limit/_maxval: Value=KOUTP_LRWheelDebug_flg_maxval
      link override Signal_Limit/_minval: Value=KOUTP_LRWheelDebug_flg_minval
      link override Signal_Override/_ovrdflg: Value=KOUTP_LRWheelDebug_flg_ovrdflg
      link override Signal_Override/_ovrdval: Value=KOUTP_LRWheelDebug_flg_ovrdval
  VTPM_LRWheelPSW_raw8_Inproc : FVT_lib/outp/OverrideAndLimit  SystemSampleTime=-1  VariantActivationTime=update diagram  Latency=0  AutoFrameSizeCalculation=off
      link override Signal_Limit/_maxval: Value=KOUTP_LRWheelPSW_raw8_maxval
      link override Signal_Limit/_minval: Value=KOUTP_LRWheelPSW_raw8_minval
      link override Signal_Override/_ovrdflg: Value=KOUTP_LRWheelPSW_raw8_ovrdflg
      link override Signal_Override/_ovrdval: Value=KOUTP_LRWheelPSW_raw8_ovrdval
  VTPM_LRWheelPress_raw8_Inproc : FVT_lib/outp/OverrideAndLimit  SystemSampleTime=-1  VariantActivationTime=update diagram  Latency=0  AutoFrameSizeCalculation=off
      link override Signal_Limit/_maxval: Value=KOUTP_LRWheelPress_raw8_maxval
      link override Signal_Limit/_minval: Value=KOUTP_LRWheelPress_raw8_minval
      link override Signal_Override/_ovrdflg: Value=KOUTP_LRWheelPress_raw8_ovrdflg
      link override Signal_Override/_ovrdval: Value=KOUTP_LRWheelPress_raw8_ovrdval
  VTPM_LRWheelTemp_C_Inproc : FVT_lib/outp/OverrideAndLimit  SystemSampleTime=-1  VariantActivationTime=update diagram  Latency=0  AutoFrameSizeCalculation=off
      link override Signal_Limit/_maxval: Value=KOUTP_LRWheelTemp_C_maxval
      link override Signal_Limit/_minval: Value=KOUTP_LRWheelTemp_C_minval
      link override Signal_Override/_ovrdflg: Value=KOUTP_LRWheelTemp_C_ovrdflg
      link override Signal_Override/_ovrdval: Value=KOUTP_LRWheelTemp_C_ovrdval
  VTPM_LRWheelTmpIndi_flg_Inproc : FVT_lib/outp/OverrideAndLimit  SystemSampleTime=-1  VariantActivationTime=update diagram  Latency=0  AutoFrameSizeCalculation=off
      link override Signal_Limit/_maxval: Value=KOUTP_LRWheelTmpIndi_flg_maxval
      link override Signal_Limit/_minval: Value=KOUTP_LRWheelTmpIndi_flg_minval
      link override Signal_Override/_ovrdflg: Value=KOUTP_LRWheelTmpIndi_flg_ovrdflg
      link override Signal_Override/_ovrdval: Value=KOUTP_LRWheelTmpIndi_flg_ovrdval
  VTPM_Prepresstempvalid_enum_Inproc : FVT_lib/outp/OverrideAndLimit  SystemSampleTime=-1  VariantActivationTime=update diagram  Latency=0  AutoFrameSizeCalculation=off
      link override Signal_Limit/_maxval: Value=KOUTP_Prepresstempvalid_enum_maxval
      link override Signal_Limit/_minval: Value=KOUTP_Prepresstempvalid_enum_minval
      link override Signal_Override/_ovrdflg: Value=KOUTP_Prepresstempvalid_enum_ovrdflg
      link override Signal_Override/_ovrdval: Value=KOUTP_Prepresstempvalid_enum_ovrdval
  VTPM_RFBatWarn_flg_Inproc : FVT_lib/outp/OverrideAndLimit  SystemSampleTime=-1  VariantActivationTime=update diagram  Latency=0  AutoFrameSizeCalculation=off
      link override Signal_Limit/_maxval: Value=KOUTP_RFBatWarn_flg_maxval
      link override Signal_Limit/_minval: Value=KOUTP_RFBatWarn_flg_minval
      link override Signal_Override/_ovrdflg: Value=KOUTP_RFBatWarn_flg_ovrdflg
      link override Signal_Override/_ovrdval: Value=KOUTP_RFBatWarn_flg_ovrdval
  VTPM_RFP20_raw8_Inproc : FVT_lib/outp/OverrideAndLimit  SystemSampleTime=-1  VariantActivationTime=update diagram  Latency=0  AutoFrameSizeCalculation=off
      link override Signal_Limit/_maxval: Value=KOUTP_RFP20_raw8_maxval
      link override Signal_Limit/_minval: Value=KOUTP_RFP20_raw8_minval
      link override Signal_Override/_ovrdflg: Value=KOUTP_RFP20_raw8_ovrdflg
      link override Signal_Override/_ovrdval: Value=KOUTP_RFP20_raw8_ovrdval
  VTPM_RFPind_enum_Inproc : FVT_lib/outp/OverrideAndLimit  SystemSampleTime=-1  VariantActivationTime=update diagram  Latency=0  AutoFrameSizeCalculation=off
      link override Signal_Limit/_maxval: Value=KOUTP_RFPind_enum_maxval
      link override Signal_Limit/_minval: Value=KOUTP_RFPind_enum_minval
      link override Signal_Override/_ovrdflg: Value=KOUTP_RFPind_enum_ovrdflg
      link override Signal_Override/_ovrdval: Value=KOUTP_RFPind_enum_ovrdval
  VTPM_RFPressIndi_enum_Inproc : FVT_lib/outp/OverrideAndLimit  SystemSampleTime=-1  VariantActivationTime=update diagram  Latency=0  AutoFrameSizeCalculation=off
      link override Signal_Limit/_maxval: Value=KOUTP_RFPressIndi_enum_maxval
      link override Signal_Limit/_minval: Value=KOUTP_RFPressIndi_enum_minval
      link override Signal_Override/_ovrdflg: Value=KOUTP_RFPressIndi_enum_ovrdflg
      link override Signal_Override/_ovrdval: Value=KOUTP_RFPressIndi_enum_ovrdval
  VTPM_RFSensorFail_flg_Inproc : FVT_lib/outp/OverrideAndLimit  SystemSampleTime=-1  VariantActivationTime=update diagram  Latency=0  AutoFrameSizeCalculation=off
      link override Signal_Limit/_maxval: Value=KOUTP_RFSensorFail_flg_maxval
      link override Signal_Limit/_minval: Value=KOUTP_RFSensorFail_flg_minval
      link override Signal_Override/_ovrdflg: Value=KOUTP_RFSensorFail_flg_ovrdflg
      link override Signal_Override/_ovrdval: Value=KOUTP_RFSensorFail_flg_ovrdval
  VTPM_RFSensorMode_flg_Inproc : FVT_lib/outp/OverrideAndLimit  SystemSampleTime=-1  VariantActivationTime=update diagram  Latency=0  AutoFrameSizeCalculation=off
      link override Signal_Limit/_maxval: Value=KOUTP_RFSensorMode_flg_maxval
      link override Signal_Limit/_minval: Value=KOUTP_RFSensorMode_flg_minval
      link override Signal_Override/_ovrdflg: Value=KOUTP_RFSensorMode_flg_ovrdflg
      link override Signal_Override/_ovrdval: Value=KOUTP_RFSensorMode_flg_ovrdval
  VTPM_RFWheelDebug_flg_Inproc : FVT_lib/outp/OverrideAndLimit  SystemSampleTime=-1  VariantActivationTime=update diagram  Latency=0  AutoFrameSizeCalculation=off
      link override Signal_Limit/_maxval: Value=KOUTP_RFWheelDebug_flg_maxval
      link override Signal_Limit/_minval: Value=KOUTP_RFWheelDebug_flg_minval
      link override Signal_Override/_ovrdflg: Value=KOUTP_RFWheelDebug_flg_ovrdflg
      link override Signal_Override/_ovrdval: Value=KOUTP_RFWheelDebug_flg_ovrdval
  VTPM_RFWheelPSW_raw8_Inproc : FVT_lib/outp/OverrideAndLimit  SystemSampleTime=-1  VariantActivationTime=update diagram  Latency=0  AutoFrameSizeCalculation=off
      link override Signal_Limit/_maxval: Value=KOUTP_RFWheelPSW_raw8_maxval
      link override Signal_Limit/_minval: Value=KOUTP_RFWheelPSW_raw8_minval
      link override Signal_Override/_ovrdflg: Value=KOUTP_RFWheelPSW_raw8_ovrdflg
      link override Signal_Override/_ovrdval: Value=KOUTP_RFWheelPSW_raw8_ovrdval
  VTPM_RFWheelPress_raw8_Inproc : FVT_lib/outp/OverrideAndLimit  SystemSampleTime=-1  VariantActivationTime=update diagram  Latency=0  AutoFrameSizeCalculation=off
      link override Signal_Limit/_maxval: Value=KOUTP_RFWheelPress_raw8_maxval
      link override Signal_Limit/_minval: Value=KOUTP_RFWheelPress_raw8_minval
      link override Signal_Override/_ovrdflg: Value=KOUTP_RFWheelPress_raw8_ovrdflg
      link override Signal_Override/_ovrdval: Value=KOUTP_RFWheelPress_raw8_ovrdval
  VTPM_RFWheelTemp_C_Inproc : FVT_lib/outp/OverrideAndLimit  SystemSampleTime=-1  VariantActivationTime=update diagram  Latency=0  AutoFrameSizeCalculation=off
      link override Signal_Limit/_maxval: Value=KOUTP_RFWheelTemp_C_maxval
      link override Signal_Limit/_minval: Value=KOUTP_RFWheelTemp_C_minval
      link override Signal_Override/_ovrdflg: Value=KOUTP_RFWheelTemp_C_ovrdflg
      link override Signal_Override/_ovrdval: Value=KOUTP_RFWheelTemp_C_ovrdval
  VTPM_RFWheelTmpIndi_flg_Inproc : FVT_lib/outp/OverrideAndLimit  SystemSampleTime=-1  VariantActivationTime=update diagram  Latency=0  AutoFrameSizeCalculation=off
      link override Signal_Limit/_maxval: Value=KOUTP_RFWheelTmpIndi_flg_maxval
      link override Signal_Limit/_minval: Value=KOUTP_RFWheelTmpIndi_flg_minval
      link override Signal_Override/_ovrdflg: Value=KOUTP_RFWheelTmpIndi_flg_ovrdflg
      link override Signal_Override/_ovrdval: Value=KOUTP_RFWheelTmpIndi_flg_ovrdval
  VTPM_RRBatWarn_flg_Inproc : FVT_lib/outp/OverrideAndLimit  SystemSampleTime=-1  VariantActivationTime=update diagram  Latency=0  AutoFrameSizeCalculation=off
      link override Signal_Limit/_maxval: Value=KOUTP_RRBatWarn_flg_maxval
      link override Signal_Limit/_minval: Value=KOUTP_RRBatWarn_flg_minval
      link override Signal_Override/_ovrdflg: Value=KOUTP_RRBatWarn_flg_ovrdflg
      link override Signal_Override/_ovrdval: Value=KOUTP_RRBatWarn_flg_ovrdval
  VTPM_RRP20_raw8_Inproc : FVT_lib/outp/OverrideAndLimit  SystemSampleTime=-1  VariantActivationTime=update diagram  Latency=0  AutoFrameSizeCalculation=off
      link override Signal_Limit/_maxval: Value=KOUTP_RRP20_raw8_maxval
      link override Signal_Limit/_minval: Value=KOUTP_RRP20_raw8_minval
      link override Signal_Override/_ovrdflg: Value=KOUTP_RRP20_raw8_ovrdflg
      link override Signal_Override/_ovrdval: Value=KOUTP_RRP20_raw8_ovrdval
  VTPM_RRPindi_enum_Inproc : FVT_lib/outp/OverrideAndLimit  SystemSampleTime=-1  VariantActivationTime=update diagram  Latency=0  AutoFrameSizeCalculation=off
      link override Signal_Limit/_maxval: Value=KOUTP_RRPindi_enum_maxval
      link override Signal_Limit/_minval: Value=KOUTP_RRPindi_enum_minval
      link override Signal_Override/_ovrdflg: Value=KOUTP_RRPindi_enum_ovrdflg
      link override Signal_Override/_ovrdval: Value=KOUTP_RRPindi_enum_ovrdval
  VTPM_RRPressIndi_enum_Inproc : FVT_lib/outp/OverrideAndLimit  SystemSampleTime=-1  VariantActivationTime=update diagram  Latency=0  AutoFrameSizeCalculation=off
      link override Signal_Limit/_maxval: Value=KOUTP_RRPressIndi_enum_maxval
      link override Signal_Limit/_minval: Value=KOUTP_RRPressIndi_enum_minval
      link override Signal_Override/_ovrdflg: Value=KOUTP_RRPressIndi_enum_ovrdflg
      link override Signal_Override/_ovrdval: Value=KOUTP_RRPressIndi_enum_ovrdval
  VTPM_RRSensorFail_flg_Inproc : FVT_lib/outp/OverrideAndLimit  SystemSampleTime=-1  VariantActivationTime=update diagram  Latency=0  AutoFrameSizeCalculation=off
      link override Signal_Limit/_maxval: Value=KOUTP_RRSensorFail_flg_maxval
      link override Signal_Limit/_minval: Value=KOUTP_RRSensorFail_flg_minval
      link override Signal_Override/_ovrdflg: Value=KOUTP_RRSensorFail_flg_ovrdflg
      link override Signal_Override/_ovrdval: Value=KOUTP_RRSensorFail_flg_ovrdval
  VTPM_RRSensorMode_flg_Inproc : FVT_lib/outp/OverrideAndLimit  SystemSampleTime=-1  VariantActivationTime=update diagram  Latency=0  AutoFrameSizeCalculation=off
      link override Signal_Limit/_maxval: Value=KOUTP_RRSensorMode_flg_maxval
      link override Signal_Limit/_minval: Value=KOUTP_RRSensorMode_flg_minval
      link override Signal_Override/_ovrdflg: Value=KOUTP_RRSensorMode_flg_ovrdflg
      link override Signal_Override/_ovrdval: Value=KOUTP_RRSensorMode_flg_ovrdval
  VTPM_RRWheelDebug_flg_Inproc : FVT_lib/outp/OverrideAndLimit  SystemSampleTime=-1  VariantActivationTime=update diagram  Latency=0  AutoFrameSizeCalculation=off
      link override Signal_Limit/_maxval: Value=KOUTP_RRWheelDebug_flg_maxval
      link override Signal_Limit/_minval: Value=KOUTP_RRWheelDebug_flg_minval
      link override Signal_Override/_ovrdflg: Value=KOUTP_RRWheelDebug_flg_ovrdflg
      link override Signal_Override/_ovrdval: Value=KOUTP_RRWheelDebug_flg_ovrdval
  VTPM_RRWheelPSW_raw8_Inproc : FVT_lib/outp/OverrideAndLimit  SystemSampleTime=-1  VariantActivationTime=update diagram  Latency=0  AutoFrameSizeCalculation=off
      link override Signal_Limit/_maxval: Value=KOUTP_RRWheelPSW_raw8_maxval
      link override Signal_Limit/_minval: Value=KOUTP_RRWheelPSW_raw8_minval
      link override Signal_Override/_ovrdflg: Value=KOUTP_RRWheelPSW_raw8_ovrdflg
      link override Signal_Override/_ovrdval: Value=KOUTP_RRWheelPSW_raw8_ovrdval
  VTPM_RRWheelPress_raw8_Inproc : FVT_lib/outp/OverrideAndLimit  SystemSampleTime=-1  VariantActivationTime=update diagram  Latency=0  AutoFrameSizeCalculation=off
      link override Signal_Limit/_maxval: Value=KOUTP_RRWheelPress_raw8_maxval
      link override Signal_Limit/_minval: Value=KOUTP_RRWheelPress_raw8_minval
      link override Signal_Override/_ovrdflg: Value=KOUTP_RRWheelPress_raw8_ovrdflg
      link override Signal_Override/_ovrdval: Value=KOUTP_RRWheelPress_raw8_ovrdval
  VTPM_RRWheelTemp_C_Inproc : FVT_lib/outp/OverrideAndLimit  SystemSampleTime=-1  VariantActivationTime=update diagram  Latency=0  AutoFrameSizeCalculation=off
      link override Signal_Limit/_maxval: Value=KOUTP_RRWheelTemp_C_maxval
      link override Signal_Limit/_minval: Value=KOUTP_RRWheelTemp_C_minval
      link override Signal_Override/_ovrdflg: Value=KOUTP_RRWheelTemp_C_ovrdflg
      link override Signal_Override/_ovrdval: Value=KOUTP_RRWheelTemp_C_ovrdval
  VTPM_RRWheelTmpIndi_flg_Inproc : FVT_lib/outp/OverrideAndLimit  SystemSampleTime=-1  VariantActivationTime=update diagram  Latency=0  AutoFrameSizeCalculation=off
      link override Signal_Limit/_maxval: Value=KOUTP_RRWheelTmpIndi_flg_maxval
      link override Signal_Limit/_minval: Value=KOUTP_RRWheelTmpIndi_flg_minval
      link override Signal_Override/_ovrdflg: Value=KOUTP_RRWheelTmpIndi_flg_ovrdflg
      link override Signal_Override/_ovrdval: Value=KOUTP_RRWheelTmpIndi_flg_ovrdval
  VTPM_S1ID_raw32_Inproc : FVT_lib/outp/OverrideAndLimit  SystemSampleTime=-1  VariantActivationTime=update diagram  Latency=0  AutoFrameSizeCalculation=off
      link override Signal_Limit/_maxval: Value=KOUTP_S1ID_raw32_maxval
      link override Signal_Limit/_minval: Value=KOUTP_S1ID_raw32_minval
      link override Signal_Override/_ovrdflg: Value=KOUTP_S1ID_raw32_ovrdflg
      link override Signal_Override/_ovrdval: Value=KOUTP_S1ID_raw32_ovrdval
  VTPM_S1L_enum_Inproc : FVT_lib/outp/OverrideAndLimit  SystemSampleTime=-1  VariantActivationTime=update diagram  Latency=0  AutoFrameSizeCalculation=off
      link override Signal_Limit/_maxval: Value=KOUTP_S1L_enum_maxval
      link override Signal_Limit/_minval: Value=KOUTP_S1L_enum_minval
      link override Signal_Override/_ovrdflg: Value=KOUTP_S1L_enum_ovrdflg
      link override Signal_Override/_ovrdval: Value=KOUTP_S1L_enum_ovrdval
  VTPM_S1WheelDebugALTU_pct_Inproc : FVT_lib/outp/OverrideAndLimit  SystemSampleTime=-1  VariantActivationTime=update diagram  Latency=0  AutoFrameSizeCalculation=off
      link override Signal_Limit/_maxval: Value=KOUTP_S1WheelDebugALTU_pct_maxval
      link override Signal_Limit/_minval: Value=KOUTP_S1WheelDebugALTU_pct_minval
      link override Signal_Override/_ovrdflg: Value=KOUTP_S1WheelDebugALTU_pct_ovrdflg
      link override Signal_Override/_ovrdval: Value=KOUTP_S1WheelDebugALTU_pct_ovrdval
  VTPM_S2ID_raw32_Inproc : FVT_lib/outp/OverrideAndLimit  SystemSampleTime=-1  VariantActivationTime=update diagram  Latency=0  AutoFrameSizeCalculation=off
      link override Signal_Limit/_maxval: Value=KOUTP_S2ID_raw32_maxval
      link override Signal_Limit/_minval: Value=KOUTP_S2ID_raw32_minval
      link override Signal_Override/_ovrdflg: Value=KOUTP_S2ID_raw32_ovrdflg
      link override Signal_Override/_ovrdval: Value=KOUTP_S2ID_raw32_ovrdval
  VTPM_S2L_enum_Inproc : FVT_lib/outp/OverrideAndLimit  SystemSampleTime=-1  VariantActivationTime=update diagram  Latency=0  AutoFrameSizeCalculation=off
      link override Signal_Limit/_maxval: Value=KOUTP_S2L_enum_maxval
      link override Signal_Limit/_minval: Value=KOUTP_S2L_enum_minval
      link override Signal_Override/_ovrdflg: Value=KOUTP_S2L_enum_ovrdflg
      link override Signal_Override/_ovrdval: Value=KOUTP_S2L_enum_ovrdval
  VTPM_S2WheelDebugALTU_pct_Inproc : FVT_lib/outp/OverrideAndLimit  SystemSampleTime=-1  VariantActivationTime=update diagram  Latency=0  AutoFrameSizeCalculation=off
      link override Signal_Limit/_maxval: Value=KOUTP_S2WheelDebugALTU_pct_maxval
      link override Signal_Limit/_minval: Value=KOUTP_S2WheelDebugALTU_pct_minval
      link override Signal_Override/_ovrdflg: Value=KOUTP_S2WheelDebugALTU_pct_ovrdflg
      link override Signal_Override/_ovrdval: Value=KOUTP_S2WheelDebugALTU_pct_ovrdval
  VTPM_S3ID_raw32_Inproc : FVT_lib/outp/OverrideAndLimit  SystemSampleTime=-1  VariantActivationTime=update diagram  Latency=0  AutoFrameSizeCalculation=off
      link override Signal_Limit/_maxval: Value=KOUTP_S3ID_raw32_maxval
      link override Signal_Limit/_minval: Value=KOUTP_S3ID_raw32_minval
      link override Signal_Override/_ovrdflg: Value=KOUTP_S3ID_raw32_ovrdflg
      link override Signal_Override/_ovrdval: Value=KOUTP_S3ID_raw32_ovrdval
  VTPM_S3L_enum_Inproc : FVT_lib/outp/OverrideAndLimit  SystemSampleTime=-1  VariantActivationTime=update diagram  Latency=0  AutoFrameSizeCalculation=off
      link override Signal_Limit/_maxval: Value=KOUTP_S3L_enum_maxval
      link override Signal_Limit/_minval: Value=KOUTP_S3L_enum_minval
      link override Signal_Override/_ovrdflg: Value=KOUTP_S3L_enum_ovrdflg
      link override Signal_Override/_ovrdval: Value=KOUTP_S3L_enum_ovrdval
  VTPM_S3WheelDebugALTU_pct_Inproc : FVT_lib/outp/OverrideAndLimit  SystemSampleTime=-1  VariantActivationTime=update diagram  Latency=0  AutoFrameSizeCalculation=off
      link override Signal_Limit/_maxval: Value=KOUTP_S3WheelDebugALTU_pct_maxval
      link override Signal_Limit/_minval: Value=KOUTP_S3WheelDebugALTU_pct_minval
      link override Signal_Override/_ovrdflg: Value=KOUTP_S3WheelDebugALTU_pct_ovrdflg
      link override Signal_Override/_ovrdval: Value=KOUTP_S3WheelDebugALTU_pct_ovrdval
